simulink library "outp"  (R2021b)
(part 7 of 11)

      link override Signal_Limit/_minval: Value=KOUTP_LimpHomeActTmp_flg_minval
      link override Signal_Override/_ovrdflg: Value=KOUTP_LimpHomeActTmp_flg_ovrdflg
      link override Signal_Override/_ovrdval: Value=KOUTP_LimpHomeActTmp_flg_ovrdval
  VDDM_Lv1ErrDTC_raw32_Inproc : FVT_lib/outp/OverrideAndLimit  SystemSampleTime=-1  VariantActivationTime=update diagram  Latency=0  AutoFrameSizeCalculation=off
      link override Signal_Limit/_maxval: Value=KOUTP_Lv1ErrDTC_raw32_maxval
      link override Signal_Limit/_minval: Value=KOUTP_Lv1ErrDTC_raw32_minval
      link override Signal_Override/_ovrdflg: Value=KOUTP_Lv1ErrDTC_raw32_ovrdflg
      link override Signal_Override/_ovrdval: Value=KOUTP_Lv1ErrDTC_raw32_ovrdval
  VDDM_Lv2ErrDTC_raw32_Inproc : FVT_lib/outp/OverrideAndLimit  SystemSampleTime=-1  VariantActivationTime=update diagram  Latency=0  AutoFrameSizeCalculation=off
      link override Signal_Limit/_maxval: Value=KOUTP_Lv2ErrDTC_raw32_maxval
      link override Signal_Limit/_minval: Value=KOUTP_Lv2ErrDTC_raw32_minval
      link override Signal_Override/_ovrdflg: Value=KOUTP_Lv2ErrDTC_raw32_ovrdflg
      link override Signal_Override/_ovrdval: Value=KOUTP_Lv2ErrDTC_raw32_ovrdval
  VDDM_Lv3ErrDTC_raw32_Inproc : FVT_lib/outp/OverrideAndLimit  SystemSampleTime=-1  VariantActivationTime=update diagram  Latency=0  AutoFrameSizeCalculation=off
      link override Signal_Limit/_maxval: Value=KOUTP_Lv3ErrDTC_raw32_maxval
      link override Signal_Limit/_minval: Value=KOUTP_Lv3ErrDTC_raw32_minval
      link override Signal_Override/_ovrdflg: Value=KOUTP_Lv3ErrDTC_raw32_ovrdflg
      link override Signal_Override/_ovrdval: Value=KOUTP_Lv3ErrDTC_raw32_ovrdval
  VDDM_Lv4ErrDTC_raw32_Inproc : FVT_lib/outp/OverrideAndLimit  SystemSampleTime=-1  VariantActivationTime=update diagram  Latency=0  AutoFrameSizeCalculation=off
      link override Signal_Limit/_maxval: Value=KOUTP_Lv4ErrDTC_raw32_maxval
      link override Signal_Limit/_minval: Value=KOUTP_Lv4ErrDTC_raw32_minval
      link override Signal_Override/_ovrdflg: Value=KOUTP_Lv4ErrDTC_raw32_ovrdflg
      link override Signal_Override/_ovrdval: Value=KOUTP_Lv4ErrDTC_raw32_ovrdval
  VDDM_MCU4PreDTC_raw32_Inproc : FVT_lib/outp/OverrideAndLimit  SystemSampleTime=-1  VariantActivationTime=update diagram  Latency=0  AutoFrameSizeCalculation=off
      link override Signal_Limit/_maxval: Value=KOUTP_MCU4PreDTC_raw32_maxval
      link override Signal_Limit/_minval: Value=KOUTP_MCU4PreDTC_raw32_minval
      link override Signal_Override/_ovrdflg: Value=KOUTP_MCU4PreDTC_raw32_ovrdflg
      link override Signal_Override/_ovrdval: Value=KOUTP_MCU4PreDTC_raw32_ovrdval
  VDDM_MCUActDTC_raw32_Inproc : FVT_lib/outp/OverrideAndLimit  SystemSampleTime=-1  VariantActivationTime=update diagram  Latency=0  AutoFrameSizeCalculation=off
      link override Signal_Limit/_maxval: Value=KOUTP_MCUActDTC_raw32_maxval
      link override Signal_Limit/_minval: Value=KOUTP_MCUActDTC_raw32_minval
      link override Signal_Override/_ovrdflg: Value=KOUTP_MCUActDTC_raw32_ovrdflg
      link override Signal_Override/_ovrdval: Value=KOUTP_MCUActDTC_raw32_ovrdval
  VDDM_MCUActDisFail_flg_Inproc : FVT_lib/outp/OverrideAndLimit  SystemSampleTime=-1  VariantActivationTime=update diagram  Latency=0  AutoFrameSizeCalculation=off
      link override Signal_Limit/_maxval: Value=KOUTP_MCUActDisFail_flg_maxval
      link override Signal_Limit/_minval: Value=KOUTP_MCUActDisFail_flg_minval
      link override Signal_Override/_ovrdflg: Value=KOUTP_MCUActDisFail_flg_ovrdflg
      link override Signal_Override/_ovrdval: Value=KOUTP_MCUActDisFail_flg_ovrdval
  VDDM_MCUDisDTC_raw32_Inproc : FVT_lib/outp/OverrideAndLimit  SystemSampleTime=-1  VariantActivationTime=update diagram  Latency=0  AutoFrameSizeCalculation=off
      link override Signal_Limit/_maxval: Value=KOUTP_MCUDisDTC_raw32_maxval
      link override Signal_Limit/_minval: Value=KOUTP_MCUDisDTC_raw32_minval
      link override Signal_Override/_ovrdflg: Value=KOUTP_MCUDisDTC_raw32_ovrdflg
      link override Signal_Override/_ovrdval: Value=KOUTP_MCUDisDTC_raw32_ovrdval
  VDDM_MCUF1CSErrDTC_raw32_Inproc : FVT_lib/outp/OverrideAndLimit  SystemSampleTime=-1  VariantActivationTime=update diagram  Latency=0  AutoFrameSizeCalculation=off
      link override Signal_Limit/_maxval: Value=KOUTP_MCUF1CSErrDTC_raw32_maxval
      link override Signal_Limit/_minval: Value=KOUTP_MCUF1CSErrDTC_raw32_minval
      link override Signal_Override/_ovrdflg: Value=KOUTP_MCUF1CSErrDTC_raw32_ovrdflg
      link override Signal_Override/_ovrdval: Value=KOUTP_MCUF1CSErrDTC_raw32_ovrdval
  VDDM_MCUF1NoComDTC_raw32_Inproc : FVT_lib/outp/OverrideAndLimit  SystemSampleTime=-1  VariantActivationTime=update diagram  Latency=0  AutoFrameSizeCalculation=off
      link override Signal_Limit/_maxval: Value=KOUTP_MCUF1NoComDTC_raw32_maxval
      link override Signal_Limit/_minval: Value=KOUTP_MCUF1NoComDTC_raw32_minval
      link override Signal_Override/_ovrdflg: Value=KOUTP_MCUF1NoComDTC_raw32_ovrdflg
      link override Signal_Override/_ovrdval: Value=KOUTP_MCUF1NoComDTC_raw32_ovrdval
  VDDM_MCUF1RCErrDTC_raw32_Inproc : FVT_lib/outp/OverrideAndLimit  SystemSampleTime=-1  VariantActivationTime=update diagram  Latency=0  AutoFrameSizeCalculation=off
      link override Signal_Limit/_maxval: Value=KOUTP_MCUF1RCErrDTC_raw32_maxval
      link override Signal_Limit/_minval: Value=KOUTP_MCUF1RCErrDTC_raw32_minval
      link override Signal_Override/_ovrdflg: Value=KOUTP_MCUF1RCErrDTC_raw32_ovrdflg
      link override Signal_Override/_ovrdval: Value=KOUTP_MCUF1RCErrDTC_raw32_ovrdval
  VDDM_MCUR1CSErrDTC_raw32_Inproc : FVT_lib/outp/OverrideAndLimit  SystemSampleTime=-1  VariantActivationTime=update diagram  Latency=0  AutoFrameSizeCalculation=off
      link override Signal_Limit/_maxval: Value=KOUTP_MCUR1CSErrDTC_raw32_maxval
      link override Signal_Limit/_minval: Value=KOUTP_MCUR1CSErrDTC_raw32_minval
      link override Signal_Override/_ovrdflg: Value=KOUTP_MCUR1CSErrDTC_raw32_ovrdflg
      link override Signal_Override/_ovrdval: Value=KOUTP_MCUR1CSErrDTC_raw32_ovrdval
  VDDM_MCUR1NoComDTC_raw32_Inproc : FVT_lib/outp/OverrideAndLimit  SystemSampleTime=-1  VariantActivationTime=update diagram  Latency=0  AutoFrameSizeCalculation=off
      link override Signal_Limit/_maxval: Value=KOUTP_MCUR1NoComDTC_raw32_maxval
      link override Signal_Limit/_minval: Value=KOUTP_MCUR1NoComDTC_raw32_minval
      link override Signal_Override/_ovrdflg: Value=KOUTP_MCUR1NoComDTC_raw32_ovrdflg
      link override Signal_Override/_ovrdval: Value=KOUTP_MCUR1NoComDTC_raw32_ovrdval
  VDDM_MCUR1RCErrDTC_raw32_Inproc : FVT_lib/outp/OverrideAndLimit  SystemSampleTime=-1  VariantActivationTime=update diagram  Latency=0  AutoFrameSizeCalculation=off
      link override Signal_Limit/_maxval: Value=KOUTP_MCUR1RCErrDTC_raw32_maxval
      link override Signal_Limit/_minval: Value=KOUTP_MCUR1RCErrDTC_raw32_minval
      link override Signal_Override/_ovrdflg: Value=KOUTP_MCUR1RCErrDTC_raw32_ovrdflg
      link override Signal_Override/_ovrdval: Value=KOUTP_MCUR1RCErrDTC_raw32_ovrdval
  VDDM_MSAMalfuncDetDTC_raw32_Inproc : FVT_lib/outp/OverrideAndLimit  SystemSampleTime=-1  VariantActivationTime=update diagram  Latency=0  AutoFrameSizeCalculation=off
      link override Signal_Limit/_maxval: Value=KOUTP_MSAMalfuncDetDTC_raw32_maxval
      link override Signal_Limit/_minval: Value=KOUTP_MSAMalfuncDetDTC_raw32_minval
      link override Signal_Override/_ovrdflg: Value=KOUTP_MSAMalfuncDetDTC_raw32_ovrdflg
      link override Signal_Override/_ovrdval: Value=KOUTP_MSAMalfuncDetDTC_raw32_ovrdval
  VDDM_MidLvSaChkDTC_raw32_Inproc : FVT_lib/outp/OverrideAndLimit  SystemSampleTime=-1  VariantActivationTime=update diagram  Latency=0  AutoFrameSizeCalculation=off
      link override Signal_Limit/_maxval: Value=KOUTP_MidLvSaChkDTC_raw32_maxval
      link override Signal_Limit/_minval: Value=KOUTP_MidLvSaChkDTC_raw32_minval
      link override Signal_Override/_ovrdflg: Value=KOUTP_MidLvSaChkDTC_raw32_ovrdflg
      link override Signal_Override/_ovrdval: Value=KOUTP_MidLvSaChkDTC_raw32_ovrdval
  VDDM_OBC4PreDTC_raw32_Inproc : FVT_lib/outp/OverrideAndLimit  SystemSampleTime=-1  VariantActivationTime=update diagram  Latency=0  AutoFrameSizeCalculation=off
      link override Signal_Limit/_maxval: Value=KOUTP_OBC4PreDTC_raw32_maxval
      link override Signal_Limit/_minval: Value=KOUTP_OBC4PreDTC_raw32_minval
      link override Signal_Override/_ovrdflg: Value=KOUTP_OBC4PreDTC_raw32_ovrdflg
      link override Signal_Override/_ovrdval: Value=KOUTP_OBC4PreDTC_raw32_ovrdval
  VDDM_ONtoRdyDTC_raw32_Inproc : FVT_lib/outp/OverrideAndLimit  SystemSampleTime=-1  VariantActivationTime=update diagram  Latency=0  AutoFrameSizeCalculation=off
      link override Signal_Limit/_maxval: Value=KOUTP_ONtoRdyDTC_raw32_maxval
      link override Signal_Limit/_minval: Value=KOUTP_ONtoRdyDTC_raw32_minval
      link override Signal_Override/_ovrdflg: Value=KOUTP_ONtoRdyDTC_raw32_ovrdflg
      link override Signal_Override/_ovrdval: Value=KOUTP_ONtoRdyDTC_raw32_ovrdval
  VDDM_RCLUSSDTC_raw32_Inproc : FVT_lib/outp/OverrideAndLimit  SystemSampleTime=-1  VariantActivationTime=update diagram  Latency=0  AutoFrameSizeCalculation=off
      link override Signal_Limit/_maxval: Value=KOUTP_RCLUSSDTC_raw32_maxval
      link override Signal_Limit/_minval: Value=KOUTP_RCLUSSDTC_raw32_minval
      link override Signal_Override/_ovrdflg: Value=KOUTP_RCLUSSDTC_raw32_ovrdflg
      link override Signal_Override/_ovrdval: Value=KOUTP_RCLUSSDTC_raw32_ovrdval
  VDDM_RCRUSSDTC_raw32_Inproc : FVT_lib/outp/OverrideAndLimit  SystemSampleTime=-1  VariantActivationTime=update diagram  Latency=0  AutoFrameSizeCalculation=off
      link override Signal_Limit/_maxval: Value=KOUTP_RCRUSSDTC_raw32_maxval
      link override Signal_Limit/_minval: Value=KOUTP_RCRUSSDTC_raw32_minval
      link override Signal_Override/_ovrdflg: Value=KOUTP_RCRUSSDTC_raw32_ovrdflg
      link override Signal_Override/_ovrdval: Value=KOUTP_RCRUSSDTC_raw32_ovrdval
  VDDM_RFBatwarnDTC_raw32_Inproc : FVT_lib/outp/OverrideAndLimit  SystemSampleTime=-1  VariantActivationTime=update diagram  Latency=0  AutoFrameSizeCalculation=off
      link override Signal_Limit/_maxval: Value=KOUTP_RFBatwarnDTC_raw32_maxval
      link override Signal_Limit/_minval: Value=KOUTP_RFBatwarnDTC_raw32_minval
      link override Signal_Override/_ovrdflg: Value=KOUTP_RFBatwarnDTC_raw32_ovrdflg
      link override Signal_Override/_ovrdval: Value=KOUTP_RFBatwarnDTC_raw32_ovrdval
  VDDM_RFPressIndiDTC_raw32_Inproc : FVT_lib/outp/OverrideAndLimit  SystemSampleTime=-1  VariantActivationTime=update diagram  Latency=0  AutoFrameSizeCalculation=off
      link override Signal_Limit/_maxval: Value=KOUTP_RFPressIndiDTC_raw32_maxval
      link override Signal_Limit/_minval: Value=KOUTP_RFPressIndiDTC_raw32_minval
      link override Signal_Override/_ovrdflg: Value=KOUTP_RFPressIndiDTC_raw32_ovrdflg
      link override Signal_Override/_ovrdval: Value=KOUTP_RFPressIndiDTC_raw32_ovrdval
  VDDM_RFSensorFailDTC_raw32_Inproc : FVT_lib/outp/OverrideAndLimit  SystemSampleTime=-1  VariantActivationTime=update diagram  Latency=0  AutoFrameSizeCalculation=off
      link override Signal_Limit/_maxval: Value=KOUTP_RFSensorFailDTC_raw32_maxval
      link override Signal_Limit/_minval: Value=KOUTP_RFSensorFailDTC_raw32_minval
      link override Signal_Override/_ovrdflg: Value=KOUTP_RFSensorFailDTC_raw32_ovrdflg
      link override Signal_Override/_ovrdval: Value=KOUTP_RFSensorFailDTC_raw32_ovrdval
  VDDM_RFWheelTmpHighDTC_raw32_Inproc : FVT_lib/outp/OverrideAndLimit  SystemSampleTime=-1  VariantActivationTime=update diagram  Latency=0  AutoFrameSizeCalculation=off
      link override Signal_Limit/_maxval: Value=KOUTP_RFWheelTmpHighDTC_raw32_maxval
      link override Signal_Limit/_minval: Value=KOUTP_RFWheelTmpHighDTC_raw32_minval
      link override Signal_Override/_ovrdflg: Value=KOUTP_RFWheelTmpHighDTC_raw32_ovrdflg
      link override Signal_Override/_ovrdval: Value=KOUTP_RFWheelTmpHighDTC_raw32_ovrdval
  VDDM_RLDoorSWDTC_raw32_Inproc : FVT_lib/outp/OverrideAndLimit  SystemSampleTime=-1  VariantActivationTime=update diagram  Latency=0  AutoFrameSizeCalculation=off
      link override Signal_Limit/_maxval: Value=KOUTP_RLDoorSWDTC_raw32_maxval
      link override Signal_Limit/_minval: Value=KOUTP_RLDoorSWDTC_raw32_minval
      link override Signal_Override/_ovrdflg: Value=KOUTP_RLDoorSWDTC_raw32_ovrdflg
      link override Signal_Override/_ovrdval: Value=KOUTP_RLDoorSWDTC_raw32_ovrdval
  VDDM_RLLUSSDTC_raw32_Inproc : FVT_lib/outp/OverrideAndLimit  SystemSampleTime=-1  VariantActivationTime=update diagram  Latency=0  AutoFrameSizeCalculation=off
      link override Signal_Limit/_maxval: Value=KOUTP_RLLUSSDTC_raw32_maxval
      link override Signal_Limit/_minval: Value=KOUTP_RLLUSSDTC_raw32_minval
      link override Signal_Override/_ovrdflg: Value=KOUTP_RLLUSSDTC_raw32_ovrdflg
      link override Signal_Override/_ovrdval: Value=KOUTP_RLLUSSDTC_raw32_ovrdval
  VDDM_RLRUSSDTC_raw32_Inproc : FVT_lib/outp/OverrideAndLimit  SystemSampleTime=-1  VariantActivationTime=update diagram  Latency=0  AutoFrameSizeCalculation=off
      link override Signal_Limit/_maxval: Value=KOUTP_RLRUSSDTC_raw32_maxval
      link override Signal_Limit/_minval: Value=KOUTP_RLRUSSDTC_raw32_minval
      link override Signal_Override/_ovrdflg: Value=KOUTP_RLRUSSDTC_raw32_ovrdflg
      link override Signal_Override/_ovrdval: Value=KOUTP_RLRUSSDTC_raw32_ovrdval
  VDDM_RMLUSSDTC_raw32_Inproc : FVT_lib/outp/OverrideAndLimit  SystemSampleTime=-1  VariantActivationTime=update diagram  Latency=0  AutoFrameSizeCalculation=off
      link override Signal_Limit/_maxval: Value=KOUTP_RMLUSSDTC_raw32_maxval
      link override Signal_Limit/_minval: Value=KOUTP_RMLUSSDTC_raw32_minval
      link override Signal_Override/_ovrdflg: Value=KOUTP_RMLUSSDTC_raw32_ovrdflg
      link override Signal_Override/_ovrdval: Value=KOUTP_RMLUSSDTC_raw32_ovrdval
  VDDM_RMRUSSDTC_raw32_Inproc : FVT_lib/outp/OverrideAndLimit  SystemSampleTime=-1  VariantActivationTime=update diagram  Latency=0  AutoFrameSizeCalculation=off
      link override Signal_Limit/_maxval: Value=KOUTP_RMRUSSDTC_raw32_maxval
      link override Signal_Limit/_minval: Value=KOUTP_RMRUSSDTC_raw32_minval
      link override Signal_Override/_ovrdflg: Value=KOUTP_RMRUSSDTC_raw32_ovrdflg
      link override Signal_Override/_ovrdval: Value=KOUTP_RMRUSSDTC_raw32_ovrdval
  VDDM_RRBatwarnDTC_raw32_Inproc : FVT_lib/outp/OverrideAndLimit  SystemSampleTime=-1  VariantActivationTime=update diagram  Latency=0  AutoFrameSizeCalculation=off
      link override Signal_Limit/_maxval: Value=KOUTP_RRBatwarnDTC_raw32_maxval
      link override Signal_Limit/_minval: Value=KOUTP_RRBatwarnDTC_raw32_minval
      link override Signal_Override/_ovrdflg: Value=KOUTP_RRBatwarnDTC_raw32_ovrdflg
      link override Signal_Override/_ovrdval: Value=KOUTP_RRBatwarnDTC_raw32_ovrdval
  VDDM_RRDoorSWDTC_raw32_Inproc : FVT_lib/outp/OverrideAndLimit  SystemSampleTime=-1  VariantActivationTime=update diagram  Latency=0  AutoFrameSizeCalculation=off
      link override Signal_Limit/_maxval: Value=KOUTP_RRDoorSWDTC_raw32_maxval
      link override Signal_Limit/_minval: Value=KOUTP_RRDoorSWDTC_raw32_minval
      link override Signal_Override/_ovrdflg: Value=KOUTP_RRDoorSWDTC_raw32_ovrdflg
      link override Signal_Override/_ovrdval: Value=KOUTP_RRDoorSWDTC_raw32_ovrdval
  VDDM_RRPressIndiDTC_raw32_Inproc : FVT_lib/outp/OverrideAndLimit  SystemSampleTime=-1  VariantActivationTime=update diagram  Latency=0  AutoFrameSizeCalculation=off
      link override Signal_Limit/_maxval: Value=KOUTP_RRPressIndiDTC_raw32_maxval
      link override Signal_Limit/_minval: Value=KOUTP_RRPressIndiDTC_raw32_minval
      link override Signal_Override/_ovrdflg: Value=KOUTP_RRPressIndiDTC_raw32_ovrdflg
      link override Signal_Override/_ovrdval: Value=KOUTP_RRPressIndiDTC_raw32_ovrdval
  VDDM_RRSensorFailDTC_raw32_Inproc : FVT_lib/outp/OverrideAndLimit  SystemSampleTime=-1  VariantActivationTime=update diagram  Latency=0  AutoFrameSizeCalculation=off
      link override Signal_Limit/_maxval: Value=KOUTP_RRSensorFailDTC_raw32_maxval
      link override Signal_Limit/_minval: Value=KOUTP_RRSensorFailDTC_raw32_minval
      link override Signal_Override/_ovrdflg: Value=KOUTP_RRSensorFailDTC_raw32_ovrdflg
      link override Signal_Override/_ovrdval: Value=KOUTP_RRSensorFailDTC_raw32_ovrdval
  VDDM_RRWheelTmpHighDTC_raw32_Inproc : FVT_lib/outp/OverrideAndLimit  SystemSampleTime=-1  VariantActivationTime=update diagram  Latency=0  AutoFrameSizeCalculation=off
      link override Signal_Limit/_maxval: Value=KOUTP_RRWheelTmpHighDTC_raw32_maxval
      link override Signal_Limit/_minval: Value=KOUTP_RRWheelTmpHighDTC_raw32_minval
      link override Signal_Override/_ovrdflg: Value=KOUTP_RRWheelTmpHighDTC_raw32_ovrdflg
      link override Signal_Override/_ovrdval: Value=KOUTP_RRWheelTmpHighDTC_raw32_ovrdval
  VDDM_RrMCUSigErrDetDTC_raw32_Inproc : FVT_lib/outp/OverrideAndLimit  SystemSampleTime=-1  VariantActivationTime=update diagram  Latency=0  AutoFrameSizeCalculation=off
      link override Signal_Limit/_maxval: Value=KOUTP_RrMCUSigErrDetDTC_raw32_maxval
      link override Signal_Limit/_minval: Value=KOUTP_RrMCUSigErrDetDTC_raw32_minval
      link override Signal_Override/_ovrdflg: Value=KOUTP_RrMCUSigErrDetDTC_raw32_ovrdflg
      link override Signal_Override/_ovrdval: Value=KOUTP_RrMCUSigErrDetDTC_raw32_ovrdval
  VDDM_RrMCUTqErrDTC_raw32_Inproc : FVT_lib/outp/OverrideAndLimit  SystemSampleTime=-1  VariantActivationTime=update diagram  Latency=0  AutoFrameSizeCalculation=off
      link override Signal_Limit/_maxval: Value=KOUTP_RrMCUTqErrDTC_raw32_maxval
      link override Signal_Limit/_minval: Value=KOUTP_RrMCUTqErrDTC_raw32_minval
      link override Signal_Override/_ovrdflg: Value=KOUTP_RrMCUTqErrDTC_raw32_ovrdflg
      link override Signal_Override/_ovrdval: Value=KOUTP_RrMCUTqErrDTC_raw32_ovrdval
  VDDM_Shifter1CSErrDTC_raw32_Inproc : FVT_lib/outp/OverrideAndLimit  SystemSampleTime=-1  VariantActivationTime=update diagram  Latency=0  AutoFrameSizeCalculation=off
      link override Signal_Limit/_maxval: Value=KOUTP_Shifter1CSErrDTC_raw32_maxval
      link override Signal_Limit/_minval: Value=KOUTP_Shifter1CSErrDTC_raw32_minval
      link override Signal_Override/_ovrdflg: Value=KOUTP_Shifter1CSErrDTC_raw32_ovrdflg
      link override Signal_Override/_ovrdval: Value=KOUTP_Shifter1CSErrDTC_raw32_ovrdval
  VDDM_Shifter1NoComDTC_raw32_Inproc : FVT_lib/outp/OverrideAndLimit  SystemSampleTime=-1  VariantActivationTime=update diagram  Latency=0  AutoFrameSizeCalculation=off
      link override Signal_Limit/_maxval: Value=KOUTP_Shifter1NoComDTC_raw32_maxval
      link override Signal_Limit/_minval: Value=KOUTP_Shifter1NoComDTC_raw32_minval
      link override Signal_Override/_ovrdflg: Value=KOUTP_Shifter1NoComDTC_raw32_ovrdflg
      link override Signal_Override/_ovrdval: Value=KOUTP_Shifter1NoComDTC_raw32_ovrdval
  VDDM_Shifter1RCErrDTC_raw32_Inproc : FVT_lib/outp/OverrideAndLimit  SystemSampleTime=-1  VariantActivationTime=update diagram  Latency=0  AutoFrameSizeCalculation=off
      link override Signal_Limit/_maxval: Value=KOUTP_Shifter1RCErrDTC_raw32_maxval
      link override Signal_Limit/_minval: Value=KOUTP_Shifter1RCErrDTC_raw32_minval
      link override Signal_Override/_ovrdflg: Value=KOUTP_Shifter1RCErrDTC_raw32_ovrdflg
      link override Signal_Override/_ovrdval: Value=KOUTP_Shifter1RCErrDTC_raw32_ovrdval
  VDDM_SysAllowReadySta_flg_Inproc : FVT_lib/outp/OverrideAndLimit  SystemSampleTime=-1  VariantActivationTime=update diagram  Latency=0  AutoFrameSizeCalculation=off
      link override Signal_Limit/_maxval: Value=KOUTP_SysAllowReadySta_flg_maxval
      link override Signal_Limit/_minval: Value=KOUTP_SysAllowReadySta_flg_minval
      link override Signal_Override/_ovrdflg: Value=KOUTP_SysAllowReadySta_flg_ovrdflg
      link override Signal_Override/_ovrdval: Value=KOUTP_SysAllowReadySta_flg_ovrdval
  VDDM_TailgaSWDTC_raw32_Inproc : FVT_lib/outp/OverrideAndLimit  SystemSampleTime=-1  VariantActivationTime=update diagram  Latency=0  AutoFrameSizeCalculation=off
      link override Signal_Limit/_maxval: Value=KOUTP_TailgaSWDTC_raw32_maxval
      link override Signal_Limit/_minval: Value=KOUTP_TailgaSWDTC_raw32_minval
      link override Signal_Override/_ovrdflg: Value=KOUTP_TailgaSWDTC_raw32_ovrdflg
      link override Signal_Override/_ovrdval: Value=KOUTP_TailgaSWDTC_raw32_ovrdval
  VDDM_VCUBrkSWSta_enum_Inproc : FVT_lib/outp/OverrideAndLimit  SystemSampleTime=-1  VariantActivationTime=update diagram  Latency=0  AutoFrameSizeCalculation=off
      link override Signal_Limit/_maxval: Value=KOUTP_VCUBrkSWSta_enum_maxval
      link override Signal_Limit/_minval: Value=KOUTP_VCUBrkSWSta_enum_minval
      link override Signal_Override/_ovrdflg: Value=KOUTP_VCUBrkSWSta_enum_ovrdflg
      link override Signal_Override/_ovrdval: Value=KOUTP_VCUBrkSWSta_enum_ovrdval
  VDDM_VCUFLDoorSta_flg_Inproc : FVT_lib/outp/OverrideAndLimit  SystemSampleTime=-1  VariantActivationTime=update diagram  Latency=0  AutoFrameSizeCalculation=off
      link override Signal_Limit/_maxval: Value=KOUTP_VCUFLDoorSta_flg_maxval
      link override Signal_Limit/_minval: Value=KOUTP_VCUFLDoorSta_flg_minval
      link override Signal_Override/_ovrdflg: Value=KOUTP_VCUFLDoorSta_flg_ovrdflg
      link override Signal_Override/_ovrdval: Value=KOUTP_VCUFLDoorSta_flg_ovrdval
  VDDM_VCUFRDoorSta_flg_Inproc : FVT_lib/outp/OverrideAndLimit  SystemSampleTime=-1  VariantActivationTime=update diagram  Latency=0  AutoFrameSizeCalculation=off
      link override Signal_Limit/_maxval: Value=KOUTP_VCUFRDoorSta_flg_maxval
      link override Signal_Limit/_minval: Value=KOUTP_VCUFRDoorSta_flg_minval
      link override Signal_Override/_ovrdflg: Value=KOUTP_VCUFRDoorSta_flg_ovrdflg
      link override Signal_Override/_ovrdval: Value=KOUTP_VCUFRDoorSta_flg_ovrdval
  VDDM_VCUHoodSWSta_flg_Inproc : FVT_lib/outp/OverrideAndLimit  SystemSampleTime=-1  VariantActivationTime=update diagram  Latency=0  AutoFrameSizeCalculation=off
      link override Signal_Limit/_maxval: Value=KOUTP_VCUHoodSWSta_flg_maxval
      link override Signal_Limit/_minval: Value=KOUTP_VCUHoodSWSta_flg_minval
      link override Signal_Override/_ovrdflg: Value=KOUTP_VCUHoodSWSta_flg_ovrdflg
      link override Signal_Override/_ovrdval: Value=KOUTP_VCUHoodSWSta_flg_ovrdval
  VDDM_VCURAPSErrLv2_flg_Inproc : FVT_lib/outp/OverrideAndLimit  SystemSampleTime=-1  VariantActivationTime=update diagram  Latency=0  AutoFrameSizeCalculation=off
      link override Signal_Limit/_maxval: Value=KOUTP_VCURAPSErrLv2_flg_maxval
      link override Signal_Limit/_minval: Value=KOUTP_VCURAPSErrLv2_flg_minval
      link override Signal_Override/_ovrdflg: Value=KOUTP_VCURAPSErrLv2_flg_ovrdflg
      link override Signal_Override/_ovrdval: Value=KOUTP_VCURAPSErrLv2_flg_ovrdval
  VDDM_VCURAPSErrLv3_flg_Inproc : FVT_lib/outp/OverrideAndLimit  SystemSampleTime=-1  VariantActivationTime=update diagram  Latency=0  AutoFrameSizeCalculation=off
      link override Signal_Limit/_maxval: Value=KOUTP_VCURAPSErrLv3_flg_maxval
      link override Signal_Limit/_minval: Value=KOUTP_VCURAPSErrLv3_flg_minval
      link override Signal_Override/_ovrdflg: Value=KOUTP_VCURAPSErrLv3_flg_ovrdflg
      link override Signal_Override/_ovrdval: Value=KOUTP_VCURAPSErrLv3_flg_ovrdval
  VDDM_VCURLDoorSta_flg_Inproc : FVT_lib/outp/OverrideAndLimit  SystemSampleTime=-1  VariantActivationTime=update diagram  Latency=0  AutoFrameSizeCalculation=off
      link override Signal_Limit/_maxval: Value=KOUTP_VCURLDoorSta_flg_maxval
      link override Signal_Limit/_minval: Value=KOUTP_VCURLDoorSta_flg_minval
      link override Signal_Override/_ovrdflg: Value=KOUTP_VCURLDoorSta_flg_ovrdflg
      link override Signal_Override/_ovrdval: Value=KOUTP_VCURLDoorSta_flg_ovrdval
  VDDM_VCURRDoorSta_flg_Inproc : FVT_lib/outp/OverrideAndLimit  SystemSampleTime=-1  VariantActivationTime=update diagram  Latency=0  AutoFrameSizeCalculation=off
      link override Signal_Limit/_maxval: Value=KOUTP_VCURRDoorSta_flg_maxval
      link override Signal_Limit/_minval: Value=KOUTP_VCURRDoorSta_flg_minval
      link override Signal_Override/_ovrdflg: Value=KOUTP_VCURRDoorSta_flg_ovrdflg
      link override Signal_Override/_ovrdval: Value=KOUTP_VCURRDoorSta_flg_ovrdval
  VDDM_VCUTailgateSWSta_flg_Inproc : FVT_lib/outp/OverrideAndLimit  SystemSampleTime=-1  VariantActivationTime=update diagram  Latency=0  AutoFrameSizeCalculation=off
      link override Signal_Limit/_maxval: Value=KOUTP_VCUTailgateSWSta_flg_maxval
      link override Signal_Limit/_minval: Value=KOUTP_VCUTailgateSWSta_flg_minval
      link override Signal_Override/_ovrdflg: Value=KOUTP_VCUTailgateSWSta_flg_ovrdflg
      link override Signal_Override/_ovrdval: Value=KOUTP_VCUTailgateSWSta_flg_ovrdval
  VDDM_VehMalfunLevel_enum_Inproc : FVT_lib/outp/OverrideAndLimit  SystemSampleTime=-1  VariantActivationTime=update diagram  Latency=0  AutoFrameSizeCalculation=off
      link override Signal_Limit/_maxval: Value=KOUTP_VehMalfunLevel_enum_maxval
      link override Signal_Limit/_minval: Value=KOUTP_VehMalfunLevel_enum_minval
      link override Signal_Override/_ovrdflg: Value=KOUTP_VehMalfunLevel_enum_ovrdflg
      link override Signal_Override/_ovrdval: Value=KOUTP_VehMalfunLevel_enum_ovrdval
  VDDM_ZoneSCPNoComDTC_raw32_Inproc : FVT_lib/outp/OverrideAndLimit  SystemSampleTime=-1  VariantActivationTime=update diagram  Latency=0  AutoFrameSizeCalculation=off
      link override Signal_Limit/_maxval: Value=KOUTP_ZoneSCPNoComDTC_raw32_maxval
      link override Signal_Limit/_minval: Value=KOUTP_ZoneSCPNoComDTC_raw32_minval
      link override Signal_Override/_ovrdflg: Value=KOUTP_ZoneSCPNoComDTC_raw32_ovrdflg
      link override Signal_Override/_ovrdval: Value=KOUTP_ZoneSCPNoComDTC_raw32_ovrdval
  VDHP_ActAPSPosn_pct_Inproc : FVT_lib/outp/OverrideAndLimit  SystemSampleTime=-1  VariantActivationTime=update diagram  Latency=0  AutoFrameSizeCalculation=off
      link override Signal_Limit/_maxval: Value=KOUTP_ActAPSPosn_pct_maxval
      link override Signal_Limit/_minval: Value=KOUTP_ActAPSPosn_pct_minval
      link override Signal_Override/_ovrdflg: Value=KOUTP_ActAPSPosn_pct_ovrdflg
      link override Signal_Override/_ovrdval: Value=KOUTP_ActAPSPosn_pct_ovrdval
  VDHP_EAPS1MIN_pct_Inproc : FVT_lib/outp/OverrideAndLimit  SystemSampleTime=-1  VariantActivationTime=update diagram  Latency=0  AutoFrameSizeCalculation=off
      link override Signal_Limit/_maxval: Value=KOUTP_EAPS1MIN_pct_maxval
      link override Signal_Limit/_minval: Value=KOUTP_EAPS1MIN_pct_minval
      link override Signal_Override/_ovrdflg: Value=KOUTP_EAPS1MIN_pct_ovrdflg
      link override Signal_Override/_ovrdval: Value=KOUTP_EAPS1MIN_pct_ovrdval
  VDHP_EAPS1NRM_pct_Inproc : FVT_lib/outp/OverrideAndLimit  SystemSampleTime=-1  VariantActivationTime=update diagram  Latency=0  AutoFrameSizeCalculation=off
      link override Signal_Limit/_maxval: Value=KOUTP_EAPS1NRM_pct_maxval
      link override Signal_Limit/_minval: Value=KOUTP_EAPS1NRM_pct_minval
      link override Signal_Override/_ovrdflg: Value=KOUTP_EAPS1NRM_pct_ovrdflg
      link override Signal_Override/_ovrdval: Value=KOUTP_EAPS1NRM_pct_ovrdval
  VDHP_EAPS2MIN_pct_Inproc : FVT_lib/outp/OverrideAndLimit  SystemSampleTime=-1  VariantActivationTime=update diagram  Latency=0  AutoFrameSizeCalculation=off
      link override Signal_Limit/_maxval: Value=KOUTP_EAPS2MIN_pct_maxval
      link override Signal_Limit/_minval: Value=KOUTP_EAPS2MIN_pct_minval
      link override Signal_Override/_ovrdflg: Value=KOUTP_EAPS2MIN_pct_ovrdflg
      link override Signal_Override/_ovrdval: Value=KOUTP_EAPS2MIN_pct_ovrdval
  VDHP_EAPS2NRM_pct_Inproc : FVT_lib/outp/OverrideAndLimit  SystemSampleTime=-1  VariantActivationTime=update diagram  Latency=0  AutoFrameSizeCalculation=off
      link override Signal_Limit/_maxval: Value=KOUTP_EAPS2NRM_pct_maxval
      link override Signal_Limit/_minval: Value=KOUTP_EAPS2NRM_pct_minval
      link override Signal_Override/_ovrdflg: Value=KOUTP_EAPS2NRM_pct_ovrdflg
      link override Signal_Override/_ovrdval: Value=KOUTP_EAPS2NRM_pct_ovrdval
  VDHP_ResetPedalZeroPosStart_flg_Inproc : FVT_lib/outp/OverrideAndLimit  SystemSampleTime=-1  VariantActivationTime=update diagram  Latency=0  AutoFrameSizeCalculation=off
      link override Signal_Limit/_maxval: Value=KOUTP_ResetPedalZeroPosStart_flg_maxval
      link override Signal_Limit/_minval: Value=KOUTP_ResetPedalZeroPosStart_flg_minval
      link override Signal_Override/_ovrdflg: Value=KOUTP_ResetPedalZeroPosStart_flg_ovrdflg
      link override Signal_Override/_ovrdval: Value=KOUTP_ResetPedalZeroPosStart_flg_ovrdval
  VDKC_DKCAuthSta_enum_Inproc : FVT_lib/outp/OverrideAndLimit  SystemSampleTime=-1  VariantActivationTime=update diagram  Latency=0  AutoFrameSizeCalculation=off
      link override Signal_Limit/_maxval: Value=KOUTP_DKCAuthSta_enum_maxval
      link override Signal_Limit/_minval: Value=KOUTP_DKCAuthSta_enum_minval
      link override Signal_Override/_ovrdflg: Value=KOUTP_DKCAuthSta_enum_ovrdflg
      link override Signal_Override/_ovrdval: Value=KOUTP_DKCAuthSta_enum_ovrdval
  VDKC_DKCTimeSN_cnt_Inproc : FVT_lib/outp/OverrideAndLimit  SystemSampleTime=-1  VariantActivationTime=update diagram  Latency=0  AutoFrameSizeCalculation=off
      link override Signal_Limit/_maxval: Value=KOUTP_DKCTimeSN_cnt_maxval
      link override Signal_Limit/_minval: Value=KOUTP_DKCTimeSN_cnt_minval
      link override Signal_Override/_ovrdflg: Value=KOUTP_DKCTimeSN_cnt_ovrdflg
      link override Signal_Override/_ovrdval: Value=KOUTP_DKCTimeSN_cnt_ovrdval
  VDKC_DKeyWelcomeSta_enum_Inproc : FVT_lib/outp/OverrideAndLimit  SystemSampleTime=-1  VariantActivationTime=update diagram  Latency=0  AutoFrameSizeCalculation=off
      link override Signal_Limit/_maxval: Value=KOUTP_DKeyWelcomeSta_enum_maxval
      link override Signal_Limit/_minval: Value=KOUTP_DKeyWelcomeSta_enum_minval
      link override Signal_Override/_ovrdflg: Value=KOUTP_DKeyWelcomeSta_enum_ovrdflg
      link override Signal_Override/_ovrdval: Value=KOUTP_DKeyWelcomeSta_enum_ovrdval
  VDKC_DkeyAreaRAPSSta_enum_Inproc : FVT_lib/outp/OverrideAndLimit  SystemSampleTime=-1  VariantActivationTime=update diagram  Latency=0  AutoFrameSizeCalculation=off
      link override Signal_Limit/_maxval: Value=KOUTP_DkeyAreaRAPSSta_enum_maxval
      link override Signal_Limit/_minval: Value=KOUTP_DkeyAreaRAPSSta_enum_minval
      link override Signal_Override/_ovrdflg: Value=KOUTP_DkeyAreaRAPSSta_enum_ovrdflg
      link override Signal_Override/_ovrdval: Value=KOUTP_DkeyAreaRAPSSta_enum_ovrdval
  VDKC_DkeyShowIVISta_enum_Inproc : FVT_lib/outp/OverrideAndLimit  SystemSampleTime=-1  VariantActivationTime=update diagram  Latency=0  AutoFrameSizeCalculation=off
      link override Signal_Limit/_maxval: Value=KOUTP_DkeyShowIVISta_enum_maxval
      link override Signal_Limit/_minval: Value=KOUTP_DkeyShowIVISta_enum_minval
      link override Signal_Override/_ovrdflg: Value=KOUTP_DkeyShowIVISta_enum_ovrdflg
      link override Signal_Override/_ovrdval: Value=KOUTP_DkeyShowIVISta_enum_ovrdval
  VDKC_FDCDKCAllowSleep_flg_Inproc : FVT_lib/outp/OverrideAndLimit  SystemSampleTime=-1  VariantActivationTime=update diagram  Latency=0  AutoFrameSizeCalculation=off
      link override Signal_Limit/_maxval: Value=KOUTP_FDCDKCAllowSleep_flg_maxval
      link override Signal_Limit/_minval: Value=KOUTP_FDCDKCAllowSleep_flg_minval
      link override Signal_Override/_ovrdflg: Value=KOUTP_FDCDKCAllowSleep_flg_ovrdflg
      link override Signal_Override/_ovrdval: Value=KOUTP_FDCDKCAllowSleep_flg_ovrdval
  VDKC_KeyAreaLockUnlock_enum_Inproc : FVT_lib/outp/OverrideAndLimit  SystemSampleTime=-1  VariantActivationTime=update diagram  Latency=0  AutoFrameSizeCalculation=off
      link override Signal_Limit/_maxval: Value=KOUTP_KeyAreaLockUnlock_enum_maxval
      link override Signal_Limit/_minval: Value=KOUTP_KeyAreaLockUnlock_enum_minval
      link override Signal_Override/_ovrdflg: Value=KOUTP_KeyAreaLockUnlock_enum_ovrdflg
      link override Signal_Override/_ovrdval: Value=KOUTP_KeyAreaLockUnlock_enum_ovrdval
  VDKC_KeyAreaPS_enum_Inproc : FVT_lib/outp/OverrideAndLimit  SystemSampleTime=-1  VariantActivationTime=update diagram  Latency=0  AutoFrameSizeCalculation=off
      link override Signal_Limit/_maxval: Value=KOUTP_KeyAreaPS_enum_maxval
      link override Signal_Limit/_minval: Value=KOUTP_KeyAreaPS_enum_minval
      link override Signal_Override/_ovrdflg: Value=KOUTP_KeyAreaPS_enum_ovrdflg
      link override Signal_Override/_ovrdval: Value=KOUTP_KeyAreaPS_enum_ovrdval
  VDKC_KeyAreaPTG_enum_Inproc : FVT_lib/outp/OverrideAndLimit  SystemSampleTime=-1  VariantActivationTime=update diagram  Latency=0  AutoFrameSizeCalculation=off
      link override Signal_Limit/_maxval: Value=KOUTP_KeyAreaPTG_enum_maxval
      link override Signal_Limit/_minval: Value=KOUTP_KeyAreaPTG_enum_minval
      link override Signal_Override/_ovrdflg: Value=KOUTP_KeyAreaPTG_enum_ovrdflg
      link override Signal_Override/_ovrdval: Value=KOUTP_KeyAreaPTG_enum_ovrdval
  VDKC_KeyAreaSPTGSta_enum_Inproc : FVT_lib/outp/OverrideAndLimit  SystemSampleTime=-1  VariantActivationTime=update diagram  Latency=0  AutoFrameSizeCalculation=off
      link override Signal_Limit/_maxval: Value=KOUTP_KeyAreaSPTGSta_enum_maxval
      link override Signal_Limit/_minval: Value=KOUTP_KeyAreaSPTGSta_enum_minval
      link override Signal_Override/_ovrdflg: Value=KOUTP_KeyAreaSPTGSta_enum_ovrdflg
      link override Signal_Override/_ovrdval: Value=KOUTP_KeyAreaSPTGSta_enum_ovrdval
  VDKC_KeyMissSta_flg_Inproc : FVT_lib/outp/OverrideAndLimit  SystemSampleTime=-1  VariantActivationTime=update diagram  Latency=0  AutoFrameSizeCalculation=off
      link override Signal_Limit/_maxval: Value=KOUTP_KeyMissSta_flg_maxval
      link override Signal_Limit/_minval: Value=KOUTP_KeyMissSta_flg_minval
      link override Signal_Override/_ovrdflg: Value=KOUTP_KeyMissSta_flg_ovrdflg
      link override Signal_Override/_ovrdval: Value=KOUTP_KeyMissSta_flg_ovrdval
  VDKC_KeyModeSta_enum_Inproc : FVT_lib/outp/OverrideAndLimit  SystemSampleTime=-1  VariantActivationTime=update diagram  Latency=0  AutoFrameSizeCalculation=off
      link override Signal_Limit/_maxval: Value=KOUTP_KeyModeSta_enum_maxval
      link override Signal_Limit/_minval: Value=KOUTP_KeyModeSta_enum_minval
      link override Signal_Override/_ovrdflg: Value=KOUTP_KeyModeSta_enum_ovrdflg
      link override Signal_Override/_ovrdval: Value=KOUTP_KeyModeSta_enum_ovrdval
  VDKC_KeyNumSta_enum_Inproc : FVT_lib/outp/OverrideAndLimit  SystemSampleTime=-1  VariantActivationTime=update diagram  Latency=0  AutoFrameSizeCalculation=off
      link override Signal_Limit/_maxval: Value=KOUTP_KeyNumSta_enum_maxval
      link override Signal_Limit/_minval: Value=KOUTP_KeyNumSta_enum_minval
      link override Signal_Override/_ovrdflg: Value=KOUTP_KeyNumSta_enum_ovrdflg
      link override Signal_Override/_ovrdval: Value=KOUTP_KeyNumSta_enum_ovrdval
  VDKC_KeyTypeSta_enum_Inproc : FVT_lib/outp/OverrideAndLimit  SystemSampleTime=-1  VariantActivationTime=update diagram  Latency=0  AutoFrameSizeCalculation=off
      link override Signal_Limit/_maxval: Value=KOUTP_KeyTypeSta_enum_maxval
      link override Signal_Limit/_minval: Value=KOUTP_KeyTypeSta_enum_minval
      link override Signal_Override/_ovrdflg: Value=KOUTP_KeyTypeSta_enum_ovrdflg
      link override Signal_Override/_ovrdval: Value=KOUTP_KeyTypeSta_enum_ovrdval
  VDKC_PCommandToBCM_enum_Inproc : FVT_lib/outp/OverrideAndLimit  SystemSampleTime=-1  VariantActivationTime=update diagram  Latency=0  AutoFrameSizeCalculation=off
      link override Signal_Limit/_maxval: Value=KOUTP_PCommandToBCM_enum_maxval
      link override Signal_Limit/_minval: Value=KOUTP_PCommandToBCM_enum_minval
      link override Signal_Override/_ovrdflg: Value=KOUTP_PCommandToBCM_enum_ovrdflg
      link override Signal_Override/_ovrdval: Value=KOUTP_PCommandToBCM_enum_ovrdval
  VDKC_ParkingModeCmd_enum_Inproc : FVT_lib/outp/OverrideAndLimit  SystemSampleTime=-1  VariantActivationTime=update diagram  Latency=0  AutoFrameSizeCalculation=off
      link override Signal_Limit/_maxval: Value=KOUTP_ParkingModeCmd_enum_maxval
      link override Signal_Limit/_minval: Value=KOUTP_ParkingModeCmd_enum_minval
      link override Signal_Override/_ovrdflg: Value=KOUTP_ParkingModeCmd_enum_ovrdflg
      link override Signal_Override/_ovrdval: Value=KOUTP_ParkingModeCmd_enum_ovrdval
  VDKC_TimeSNDKCFbk_cnt_Inproc : FVT_lib/outp/OverrideAndLimit  SystemSampleTime=-1  VariantActivationTime=update diagram  Latency=0  AutoFrameSizeCalculation=off
      link override Signal_Limit/_maxval: Value=KOUTP_TimeSNDKCFbk_cnt_maxval
      link override Signal_Limit/_minval: Value=KOUTP_TimeSNDKCFbk_cnt_minval
      link override Signal_Override/_ovrdflg: Value=KOUTP_TimeSNDKCFbk_cnt_ovrdflg
      link override Signal_Override/_ovrdval: Value=KOUTP_TimeSNDKCFbk_cnt_ovrdval
  VDKC_UIDLowPowerSta_enum_Inproc : FVT_lib/outp/OverrideAndLimit  SystemSampleTime=-1  VariantActivationTime=update diagram  Latency=0  AutoFrameSizeCalculation=off
      link override Signal_Limit/_maxval: Value=KOUTP_UIDLowPowerSta_enum_maxval
      link override Signal_Limit/_minval: Value=KOUTP_UIDLowPowerSta_enum_minval
      link override Signal_Override/_ovrdflg: Value=KOUTP_UIDLowPowerSta_enum_ovrdflg
      link override Signal_Override/_ovrdval: Value=KOUTP_UIDLowPowerSta_enum_ovrdval
  VDSC_DISCButtSta_flg_Inproc : FVT_lib/outp/OverrideAndLimit  SystemSampleTime=-1  VariantActivationTime=update diagram  Latency=0  AutoFrameSizeCalculation=off
      link override Signal_Limit/_maxval: Value=KOUTP_DISCButtSta_flg_maxval
      link override Signal_Limit/_minval: Value=KOUTP_DISCButtSta_flg_minval
      link override Signal_Override/_ovrdflg: Value=KOUTP_DISCButtSta_flg_ovrdflg
      link override Signal_Override/_ovrdval: Value=KOUTP_DISCButtSta_flg_ovrdval
  VDSC_DISCSta_enum_Inproc : FVT_lib/outp/OverrideAndLimit  SystemSampleTime=-1  VariantActivationTime=update diagram  Latency=0  AutoFrameSizeCalculation=off
      link override Signal_Limit/_maxval: Value=KOUTP_DISCSta_enum_maxval
      link override Signal_Limit/_minval: Value=KOUTP_DISCSta_enum_minval
      link override Signal_Override/_ovrdflg: Value=KOUTP_DISCSta_enum_ovrdflg
      link override Signal_Override/_ovrdval: Value=KOUTP_DISCSta_enum_ovrdval
  VDSC_DISCTargetSpd_kph_Inproc : FVT_lib/outp/OverrideAndLimit  SystemSampleTime=-1  VariantActivationTime=update diagram  Latency=0  AutoFrameSizeCalculation=off
      link override Signal_Limit/_maxval: Value=KOUTP_DISCTargetSpd_kph_maxval
      link override Signal_Limit/_minval: Value=KOUTP_DISCTargetSpd_kph_minval
      link override Signal_Override/_ovrdflg: Value=KOUTP_DISCTargetSpd_kph_ovrdflg
      link override Signal_Override/_ovrdval: Value=KOUTP_DISCTargetSpd_kph_ovrdval
  VDSC_DISCTurn_flg_Inproc : FVT_lib/outp/OverrideAndLimit  SystemSampleTime=-1  VariantActivationTime=update diagram  Latency=0  AutoFrameSizeCalculation=off
      link override Signal_Limit/_maxval: Value=KOUTP_DISCTurn_flg_maxval
      link override Signal_Limit/_minval: Value=KOUTP_DISCTurn_flg_minval
      link override Signal_Override/_ovrdflg: Value=KOUTP_DISCTurn_flg_ovrdflg
      link override Signal_Override/_ovrdval: Value=KOUTP_DISCTurn_flg_ovrdval
  VNMM_ActiveWU_flg_Inproc : FVT_lib/outp/OverrideAndLimit  SystemSampleTime=-1  VariantActivationTime=update diagram  Latency=0  AutoFrameSizeCalculation=off
      link override Signal_Limit/_maxval: Value=KOUTP_ActiveWU_flg_maxval
      link override Signal_Limit/_minval: Value=KOUTP_ActiveWU_flg_minval
      link override Signal_Override/_ovrdflg: Value=KOUTP_ActiveWU_flg_ovrdflg
      link override Signal_Override/_ovrdval: Value=KOUTP_ActiveWU_flg_ovrdval
  VNMM_AllCANTxReq_flg_Inproc : FVT_lib/outp/OverrideAndLimit  SystemSampleTime=-1  VariantActivationTime=update diagram  Latency=0  AutoFrameSizeCalculation=off
      link override Signal_Limit/_maxval: Value=KOUTP_AllCANTxReq_flg_maxval
      link override Signal_Limit/_minval: Value=KOUTP_AllCANTxReq_flg_minval
      link override Signal_Override/_ovrdflg: Value=KOUTP_AllCANTxReq_flg_ovrdflg
      link override Signal_Override/_ovrdval: Value=KOUTP_AllCANTxReq_flg_ovrdval
  VNMM_Awake_enum_Inproc : FVT_lib/outp/OverrideAndLimit  SystemSampleTime=-1  VariantActivationTime=update diagram  Latency=0  AutoFrameSizeCalculation=off
      link override Signal_Limit/_maxval: Value=KOUTP_Awake_enum_maxval
      link override Signal_Limit/_minval: Value=KOUTP_Awake_enum_minval
      link override Signal_Override/_ovrdflg: Value=KOUTP_Awake_enum_ovrdflg
      link override Signal_Override/_ovrdval: Value=KOUTP_Awake_enum_ovrdval
  VNMM_CSB_flg_Inproc : FVT_lib/outp/OverrideAndLimit  SystemSampleTime=-1  VariantActivationTime=update diagram  Latency=0  AutoFrameSizeCalculation=off
      link override Signal_Limit/_maxval: Value=KOUTP_CSB_flg_maxval
      link override Signal_Limit/_minval: Value=KOUTP_CSB_flg_minval
      link override Signal_Override/_ovrdflg: Value=KOUTP_CSB_flg_ovrdflg
      link override Signal_Override/_ovrdval: Value=KOUTP_CSB_flg_ovrdval
  VNMM_ErrorState_enum_Inproc : FVT_lib/outp/OverrideAndLimit  SystemSampleTime=-1  VariantActivationTime=update diagram  Latency=0  AutoFrameSizeCalculation=off
      link override Signal_Limit/_maxval: Value=KOUTP_ErrorState_enum_maxval
      link override Signal_Limit/_minval: Value=KOUTP_ErrorState_enum_minval
      link override Signal_Override/_ovrdflg: Value=KOUTP_ErrorState_enum_ovrdflg
      link override Signal_Override/_ovrdval: Value=KOUTP_ErrorState_enum_ovrdval
  VNMM_NMmTxReq_flg_Inproc : FVT_lib/outp/OverrideAndLimit  SystemSampleTime=-1  VariantActivationTime=update diagram  Latency=0  AutoFrameSizeCalculation=off
      link override Signal_Limit/_maxval: Value=KOUTP_NMmTxReq_flg_maxval
      link override Signal_Limit/_minval: Value=KOUTP_NMmTxReq_flg_minval
      link override Signal_Override/_ovrdflg: Value=KOUTP_NMmTxReq_flg_ovrdflg
      link override Signal_Override/_ovrdval: Value=KOUTP_NMmTxReq_flg_ovrdval
  VNMM_NetworkReq_flg_Inproc : FVT_lib/outp/OverrideAndLimit  SystemSampleTime=-1  VariantActivationTime=update diagram  Latency=0  AutoFrameSizeCalculation=off
      link override Signal_Limit/_maxval: Value=KOUTP_NetworkReq_flg_maxval
      link override Signal_Limit/_minval: Value=KOUTP_NetworkReq_flg_minval
      link override Signal_Override/_ovrdflg: Value=KOUTP_NetworkReq_flg_ovrdflg
      link override Signal_Override/_ovrdval: Value=KOUTP_NetworkReq_flg_ovrdval
  VNMM_NodeID_enum_Inproc : FVT_lib/outp/OverrideAndLimit  SystemSampleTime=-1  VariantActivationTime=update diagram  Latency=0  AutoFrameSizeCalculation=off
      link override Signal_Limit/_maxval: Value=KOUTP_NodeID_enum_maxval
      link override Signal_Limit/_minval: Value=KOUTP_NodeID_enum_minval
      link override Signal_Override/_ovrdflg: Value=KOUTP_NodeID_enum_ovrdflg
      link override Signal_Override/_ovrdval: Value=KOUTP_NodeID_enum_ovrdval
  VNMM_PNI_flg_Inproc : FVT_lib/outp/OverrideAndLimit  SystemSampleTime=-1  VariantActivationTime=update diagram  Latency=0  AutoFrameSizeCalculation=off
      link override Signal_Limit/_maxval: Value=KOUTP_PNI_flg_maxval
      link override Signal_Limit/_minval: Value=KOUTP_PNI_flg_minval
      link override Signal_Override/_ovrdflg: Value=KOUTP_PNI_flg_ovrdflg
      link override Signal_Override/_ovrdval: Value=KOUTP_PNI_flg_ovrdval
  VNMM_RptMsgReq_flg_Inproc : FVT_lib/outp/OverrideAndLimit  SystemSampleTime=-1  VariantActivationTime=update diagram  Latency=0  AutoFrameSizeCalculation=off
      link override Signal_Limit/_maxval: Value=KOUTP_RptMsgReq_flg_maxval
      link override Signal_Limit/_minval: Value=KOUTP_RptMsgReq_flg_minval
      link override Signal_Override/_ovrdflg: Value=KOUTP_RptMsgReq_flg_ovrdflg
      link override Signal_Override/_ovrdval: Value=KOUTP_RptMsgReq_flg_ovrdval
  VNMM_SysNMmSta_enum_Inproc : FVT_lib/outp/OverrideAndLimit  SystemSampleTime=-1  VariantActivationTime=update diagram  Latency=0  AutoFrameSizeCalculation=off
      link override Signal_Limit/_maxval: Value=KOUTP_SysNMmSta_enum_maxval
      link override Signal_Limit/_minval: Value=KOUTP_SysNMmSta_enum_minval
      link override Signal_Override/_ovrdflg: Value=KOUTP_SysNMmSta_enum_ovrdflg
      link override Signal_Override/_ovrdval: Value=KOUTP_SysNMmSta_enum_ovrdval
  VNMM_WakeUp_enum_Inproc : FVT_lib/outp/OverrideAndLimit  SystemSampleTime=-1  VariantActivationTime=update diagram  Latency=0  AutoFrameSizeCalculation=off
      link override Signal_Limit/_maxval: Value=KOUTP_WakeUp_enum_maxval
      link override Signal_Limit/_minval: Value=KOUTP_WakeUp_enum_minval
      link override Signal_Override/_ovrdflg: Value=KOUTP_WakeUp_enum_ovrdflg
      link override Signal_Override/_ovrdval: Value=KOUTP_WakeUp_enum_ovrdval
  VPMM_ActiveDischargeReq_flg_Inproc : FVT_lib/outp/OverrideAndLimit  SystemSampleTime=-1  VariantActivationTime=update diagram  Latency=0  AutoFrameSizeCalculation=off
      link override Signal_Limit/_maxval: Value=KOUTP_ActiveDischargeReq_flg_maxval
      link override Signal_Limit/_minval: Value=KOUTP_ActiveDischargeReq_flg_minval
      link override Signal_Override/_ovrdflg: Value=KOUTP_ActiveDischargeReq_flg_ovrdflg
      link override Signal_Override/_ovrdval: Value=KOUTP_ActiveDischargeReq_flg_ovrdval
  VPMM_CtrlDrPwrStbA2_flg_Inproc : FVT_lib/outp/OverrideAndLimit  SystemSampleTime=-1  VariantActivationTime=update diagram  Latency=0  AutoFrameSizeCalculation=off
      link override Signal_Limit/_maxval: Value=KOUTP_CtrlDrPwrStbA2_flg_maxval
      link override Signal_Limit/_minval: Value=KOUTP_CtrlDrPwrStbA2_flg_minval
      link override Signal_Override/_ovrdflg: Value=KOUTP_CtrlDrPwrStbA2_flg_ovrdflg
      link override Signal_Override/_ovrdval: Value=KOUTP_CtrlDrPwrStbA2_flg_ovrdval
  VPMM_CtrlFrBMSCCUCIR_flg_Inproc : FVT_lib/outp/OverrideAndLimit  SystemSampleTime=-1  VariantActivationTime=update diagram  Latency=0  AutoFrameSizeCalculation=off
      link override Signal_Limit/_maxval: Value=KOUTP_CtrlFrBMSCCUCIR_flg_maxval
      link override Signal_Limit/_minval: Value=KOUTP_CtrlFrBMSCCUCIR_flg_minval
      link override Signal_Override/_ovrdflg: Value=KOUTP_CtrlFrBMSCCUCIR_flg_ovrdflg
      link override Signal_Override/_ovrdval: Value=KOUTP_CtrlFrBMSCCUCIR_flg_ovrdval
  VPMM_CtrlFrEDUINVERTER_flg_Inproc : FVT_lib/outp/OverrideAndLimit  SystemSampleTime=-1  VariantActivationTime=update diagram  Latency=0  AutoFrameSizeCalculation=off
      link override Signal_Limit/_maxval: Value=KOUTP_CtrlFrEDUINVERTER_flg_maxval
      link override Signal_Limit/_minval: Value=KOUTP_CtrlFrEDUINVERTER_flg_minval
      link override Signal_Override/_ovrdflg: Value=KOUTP_CtrlFrEDUINVERTER_flg_ovrdflg
      link override Signal_Override/_ovrdval: Value=KOUTP_CtrlFrEDUINVERTER_flg_ovrdval
  VPMM_CtrlFrPwrStbA1P_flg_Inproc : FVT_lib/outp/OverrideAndLimit  SystemSampleTime=-1  VariantActivationTime=update diagram  Latency=0  AutoFrameSizeCalculation=off
      link override Signal_Limit/_maxval: Value=KOUTP_CtrlFrPwrStbA1P_flg_maxval
      link override Signal_Limit/_minval: Value=KOUTP_CtrlFrPwrStbA1P_flg_minval
      link override Signal_Override/_ovrdflg: Value=KOUTP_CtrlFrPwrStbA1P_flg_ovrdflg
      link override Signal_Override/_ovrdval: Value=KOUTP_CtrlFrPwrStbA1P_flg_ovrdval
  VPMM_CtrlFrRC1_flg_Inproc : FVT_lib/outp/OverrideAndLimit  SystemSampleTime=-1  VariantActivationTime=update diagram  Latency=0  AutoFrameSizeCalculation=off
      link override Signal_Limit/_maxval: Value=KOUTP_CtrlFrRC1_flg_maxval
      link override Signal_Limit/_minval: Value=KOUTP_CtrlFrRC1_flg_minval
      link override Signal_Override/_ovrdflg: Value=KOUTP_CtrlFrRC1_flg_ovrdflg
      link override Signal_Override/_ovrdval: Value=KOUTP_CtrlFrRC1_flg_ovrdval
  VPMM_DCDCEnaReq_flg_Inproc : FVT_lib/outp/OverrideAndLimit  SystemSampleTime=-1  VariantActivationTime=update diagram  Latency=0  AutoFrameSizeCalculation=off
      link override Signal_Limit/_maxval: Value=KOUTP_DCDCEnaReq_flg_maxval
      link override Signal_Limit/_minval: Value=KOUTP_DCDCEnaReq_flg_minval
      link override Signal_Override/_ovrdflg: Value=KOUTP_DCDCEnaReq_flg_ovrdflg
      link override Signal_Override/_ovrdval: Value=KOUTP_DCDCEnaReq_flg_ovrdval
  VPMM_DCDCVoltSetpoint_V_Inproc : FVT_lib/outp/OverrideAndLimit  SystemSampleTime=-1  VariantActivationTime=update diagram  Latency=0  AutoFrameSizeCalculation=off
      link override Signal_Limit/_maxval: Value=KOUTP_DCDCVoltSetpoint_V_maxval
      link override Signal_Limit/_minval: Value=KOUTP_DCDCVoltSetpoint_V_minval
      link override Signal_Override/_ovrdflg: Value=KOUTP_DCDCVoltSetpoint_V_ovrdflg
      link override Signal_Override/_ovrdval: Value=KOUTP_DCDCVoltSetpoint_V_ovrdval
  VPMM_DrSeatSta_enum_Inproc : FVT_lib/outp/OverrideAndLimit  SystemSampleTime=-1  VariantActivationTime=update diagram  Latency=0  AutoFrameSizeCalculation=off
      link override Signal_Limit/_maxval: Value=KOUTP_DrSeatSta_enum_maxval
      link override Signal_Limit/_minval: Value=KOUTP_DrSeatSta_enum_minval
      link override Signal_Override/_ovrdflg: Value=KOUTP_DrSeatSta_enum_ovrdflg
      link override Signal_Override/_ovrdval: Value=KOUTP_DrSeatSta_enum_ovrdval
  VPMM_DrivetrainSelect_enum_Inproc : FVT_lib/outp/OverrideAndLimit  SystemSampleTime=-1  VariantActivationTime=update diagram  Latency=0  AutoFrameSizeCalculation=off
      link override Signal_Limit/_maxval: Value=KOUTP_DrivetrainSelect_enum_maxval
      link override Signal_Limit/_minval: Value=KOUTP_DrivetrainSelect_enum_minval
      link override Signal_Override/_ovrdflg: Value=KOUTP_DrivetrainSelect_enum_ovrdflg
      link override Signal_Override/_ovrdval: Value=KOUTP_DrivetrainSelect_enum_ovrdval
  VPMM_EvccAplusPwrUpReq_flg_Inproc : FVT_lib/outp/OverrideAndLimit  SystemSampleTime=-1  VariantActivationTime=update diagram  Latency=0  AutoFrameSizeCalculation=off
      link override Signal_Limit/_maxval: Value=KOUTP_EvccAplusPwrUpReq_flg_maxval
      link override Signal_Limit/_minval: Value=KOUTP_EvccAplusPwrUpReq_flg_minval
      link override Signal_Override/_ovrdflg: Value=KOUTP_EvccAplusPwrUpReq_flg_ovrdflg
      link override Signal_Override/_ovrdval: Value=KOUTP_EvccAplusPwrUpReq_flg_ovrdval
  VPMM_FDADC12VDetAvg_mV_Inproc : FVT_lib/outp/OverrideAndLimit  SystemSampleTime=-1  VariantActivationTime=update diagram  Latency=0  AutoFrameSizeCalculation=off
      link override Signal_Limit/_maxval: Value=KOUTP_FDADC12VDetAvg_mV_maxval
      link override Signal_Limit/_minval: Value=KOUTP_FDADC12VDetAvg_mV_minval
      link override Signal_Override/_ovrdflg: Value=KOUTP_FDADC12VDetAvg_mV_ovrdflg
      link override Signal_Override/_ovrdval: Value=KOUTP_FDADC12VDetAvg_mV_ovrdval
  VPMM_FrMCUEnaReq_flg_Inproc : FVT_lib/outp/OverrideAndLimit  SystemSampleTime=-1  VariantActivationTime=update diagram  Latency=0  AutoFrameSizeCalculation=off
      link override Signal_Limit/_maxval: Value=KOUTP_FrMCUEnaReq_flg_maxval
      link override Signal_Limit/_minval: Value=KOUTP_FrMCUEnaReq_flg_minval
      link override Signal_Override/_ovrdflg: Value=KOUTP_FrMCUEnaReq_flg_ovrdflg
      link override Signal_Override/_ovrdval: Value=KOUTP_FrMCUEnaReq_flg_ovrdval
  VPMM_HVBatCnctReq_flg_Inproc : FVT_lib/outp/OverrideAndLimit  SystemSampleTime=-1  VariantActivationTime=update diagram  Latency=0  AutoFrameSizeCalculation=off
      link override Signal_Limit/_maxval: Value=KOUTP_HVBatCnctReq_flg_maxval
      link override Signal_Limit/_minval: Value=KOUTP_HVBatCnctReq_flg_minval
      link override Signal_Override/_ovrdflg: Value=KOUTP_HVBatCnctReq_flg_ovrdflg
      link override Signal_Override/_ovrdval: Value=KOUTP_HVBatCnctReq_flg_ovrdval
  VPMM_HVPwrSta_flg_Inproc : FVT_lib/outp/OverrideAndLimit  SystemSampleTime=-1  VariantActivationTime=update diagram  Latency=0  AutoFrameSizeCalculation=off
      link override Signal_Limit/_maxval: Value=KOUTP_HVPwrSta_flg_maxval
      link override Signal_Limit/_minval: Value=KOUTP_HVPwrSta_flg_minval
      link override Signal_Override/_ovrdflg: Value=KOUTP_HVPwrSta_flg_ovrdflg
      link override Signal_Override/_ovrdval: Value=KOUTP_HVPwrSta_flg_ovrdval
  VPMM_HVSysReadyToCharge_enum_Inproc : FVT_lib/outp/OverrideAndLimit  SystemSampleTime=-1  VariantActivationTime=update diagram  Latency=0  AutoFrameSizeCalculation=off
      link override Signal_Limit/_maxval: Value=KOUTP_HVSysReadyToCharge_enum_maxval
      link override Signal_Limit/_minval: Value=KOUTP_HVSysReadyToCharge_enum_minval
      link override Signal_Override/_ovrdflg: Value=KOUTP_HVSysReadyToCharge_enum_ovrdflg
      link override Signal_Override/_ovrdval: Value=KOUTP_HVSysReadyToCharge_enum_ovrdval
  VPMM_HWResetSta_enum_Inproc : FVT_lib/outp/OverrideAndLimit  SystemSampleTime=-1  VariantActivationTime=update diagram  Latency=0  AutoFrameSizeCalculation=off
      link override Signal_Limit/_maxval: Value=KOUTP_HWResetSta_enum_maxval
      link override Signal_Limit/_minval: Value=KOUTP_HWResetSta_enum_minval
      link override Signal_Override/_ovrdflg: Value=KOUTP_HWResetSta_enum_ovrdflg
      link override Signal_Override/_ovrdval: Value=KOUTP_HWResetSta_enum_ovrdval
  VPMM_IVIPwrStaONTOPopT_s_Inproc : FVT_lib/outp/OverrideAndLimit  SystemSampleTime=-1  VariantActivationTime=update diagram  Latency=0  AutoFrameSizeCalculation=off
      link override Signal_Limit/_maxval: Value=KOUTP_IVIPwrStaONTOPopT_s_maxval
      link override Signal_Limit/_minval: Value=KOUTP_IVIPwrStaONTOPopT_s_minval
      link override Signal_Override/_ovrdflg: Value=KOUTP_IVIPwrStaONTOPopT_s_ovrdflg
      link override Signal_Override/_ovrdval: Value=KOUTP_IVIPwrStaONTOPopT_s_ovrdval
  VPMM_LVBattChrgTimeCnt_s_Inproc : FVT_lib/outp/OverrideAndLimit  SystemSampleTime=-1  VariantActivationTime=update diagram  Latency=0  AutoFrameSizeCalculation=off
      link override Signal_Limit/_maxval: Value=KOUTP_LVBattChrgTimeCnt_s_maxval
      link override Signal_Limit/_minval: Value=KOUTP_LVBattChrgTimeCnt_s_minval
      link override Signal_Override/_ovrdflg: Value=KOUTP_LVBattChrgTimeCnt_s_ovrdflg
      link override Signal_Override/_ovrdval: Value=KOUTP_LVBattChrgTimeCnt_s_ovrdval
  VPMM_LVChrgHoldTtimer_s_Inproc : FVT_lib/outp/OverrideAndLimit  SystemSampleTime=-1  VariantActivationTime=update diagram  Latency=0  AutoFrameSizeCalculation=off
      link override Signal_Limit/_maxval: Value=KOUTP_LVChrgHoldTtimer_s_maxval
      link override Signal_Limit/_minval: Value=KOUTP_LVChrgHoldTtimer_s_minval
      link override Signal_Override/_ovrdflg: Value=KOUTP_LVChrgHoldTtimer_s_ovrdflg
      link override Signal_Override/_ovrdval: Value=KOUTP_LVChrgHoldTtimer_s_ovrdval
  VPMM_LVPwrSta_flg_Inproc : FVT_lib/outp/OverrideAndLimit  SystemSampleTime=-1  VariantActivationTime=update diagram  Latency=0  AutoFrameSizeCalculation=off
      link override Signal_Limit/_maxval: Value=KOUTP_LVPwrSta_flg_maxval
      link override Signal_Limit/_minval: Value=KOUTP_LVPwrSta_flg_minval
      link override Signal_Override/_ovrdflg: Value=KOUTP_LVPwrSta_flg_ovrdflg
      link override Signal_Override/_ovrdval: Value=KOUTP_LVPwrSta_flg_ovrdval
  VPMM_LVSilentChrgLv_enum_Inproc : FVT_lib/outp/OverrideAndLimit  SystemSampleTime=-1  VariantActivationTime=update diagram  Latency=0  AutoFrameSizeCalculation=off
      link override Signal_Limit/_maxval: Value=KOUTP_LVSilentChrgLv_enum_maxval
      link override Signal_Limit/_minval: Value=KOUTP_LVSilentChrgLv_enum_minval
      link override Signal_Override/_ovrdflg: Value=KOUTP_LVSilentChrgLv_enum_ovrdflg
      link override Signal_Override/_ovrdval: Value=KOUTP_LVSilentChrgLv_enum_ovrdval
  VPMM_LVSilentChrgReq_flg_Inproc : FVT_lib/outp/OverrideAndLimit  SystemSampleTime=-1  VariantActivationTime=update diagram  Latency=0  AutoFrameSizeCalculation=off
      link override Signal_Limit/_maxval: Value=KOUTP_LVSilentChrgReq_flg_maxval
      link override Signal_Limit/_minval: Value=KOUTP_LVSilentChrgReq_flg_minval
      link override Signal_Override/_ovrdflg: Value=KOUTP_LVSilentChrgReq_flg_ovrdflg
      link override Signal_Override/_ovrdval: Value=KOUTP_LVSilentChrgReq_flg_ovrdval
  VPMM_LVSilentChrgSta_enum_Inproc : FVT_lib/outp/OverrideAndLimit  SystemSampleTime=-1  VariantActivationTime=update diagram  Latency=0  AutoFrameSizeCalculation=off
      link override Signal_Limit/_maxval: Value=KOUTP_LVSilentChrgSta_enum_maxval
      link override Signal_Limit/_minval: Value=KOUTP_LVSilentChrgSta_enum_minval
      link override Signal_Override/_ovrdflg: Value=KOUTP_LVSilentChrgSta_enum_ovrdflg
      link override Signal_Override/_ovrdval: Value=KOUTP_LVSilentChrgSta_enum_ovrdval
  VPMM_LowSOCWarn_enum_Inproc : FVT_lib/outp/OverrideAndLimit  SystemSampleTime=-1  VariantActivationTime=update diagram  Latency=0  AutoFrameSizeCalculation=off
      link override Signal_Limit/_maxval: Value=KOUTP_LowSOCWarn_enum_maxval
      link override Signal_Limit/_minval: Value=KOUTP_LowSOCWarn_enum_minval
      link override Signal_Override/_ovrdflg: Value=KOUTP_LowSOCWarn_enum_ovrdflg
      link override Signal_Override/_ovrdval: Value=KOUTP_LowSOCWarn_enum_ovrdval
  VPMM_OTAPwrReqOFFChkSta_enum_Inproc : FVT_lib/outp/OverrideAndLimit  SystemSampleTime=-1  VariantActivationTime=update diagram  Latency=0  AutoFrameSizeCalculation=off
      link override Signal_Limit/_maxval: Value=KOUTP_OTAPwrReqOFFChkSta_enum_maxval
      link override Signal_Limit/_minval: Value=KOUTP_OTAPwrReqOFFChkSta_enum_minval
      link override Signal_Override/_ovrdflg: Value=KOUTP_OTAPwrReqOFFChkSta_enum_ovrdflg
      link override Signal_Override/_ovrdval: Value=KOUTP_OTAPwrReqOFFChkSta_enum_ovrdval
  VPMM_OTAPwrReqStdChkSta_enum_Inproc : FVT_lib/outp/OverrideAndLimit  SystemSampleTime=-1  VariantActivationTime=update diagram  Latency=0  AutoFrameSizeCalculation=off
      link override Signal_Limit/_maxval: Value=KOUTP_OTAPwrReqStdChkSta_enum_maxval
      link override Signal_Limit/_minval: Value=KOUTP_OTAPwrReqStdChkSta_enum_minval
      link override Signal_Override/_ovrdflg: Value=KOUTP_OTAPwrReqStdChkSta_enum_ovrdflg
      link override Signal_Override/_ovrdval: Value=KOUTP_OTAPwrReqStdChkSta_enum_ovrdval
  VPMM_PMMAllowECUSleep_flg_Inproc : FVT_lib/outp/OverrideAndLimit  SystemSampleTime=-1  VariantActivationTime=update diagram  Latency=0  AutoFrameSizeCalculation=off
      link override Signal_Limit/_maxval: Value=KOUTP_PMMAllowECUSleep_flg_maxval
      link override Signal_Limit/_minval: Value=KOUTP_PMMAllowECUSleep_flg_minval
      link override Signal_Override/_ovrdflg: Value=KOUTP_PMMAllowECUSleep_flg_ovrdflg
      link override Signal_Override/_ovrdval: Value=KOUTP_PMMAllowECUSleep_flg_ovrdval
  VPMM_PowerDownFault_enum_Inproc : FVT_lib/outp/OverrideAndLimit  SystemSampleTime=-1  VariantActivationTime=update diagram  Latency=0  AutoFrameSizeCalculation=off
      link override Signal_Limit/_maxval: Value=KOUTP_PowerDownFault_enum_maxval
      link override Signal_Limit/_minval: Value=KOUTP_PowerDownFault_enum_minval
      link override Signal_Override/_ovrdflg: Value=KOUTP_PowerDownFault_enum_ovrdflg
      link override Signal_Override/_ovrdval: Value=KOUTP_PowerDownFault_enum_ovrdval
  VPMM_PowerDownState_enum_Inproc : FVT_lib/outp/OverrideAndLimit  SystemSampleTime=-1  VariantActivationTime=update diagram  Latency=0  AutoFrameSizeCalculation=off
      link override Signal_Limit/_maxval: Value=KOUTP_PowerDownState_enum_maxval
      link override Signal_Limit/_minval: Value=KOUTP_PowerDownState_enum_minval
      link override Signal_Override/_ovrdflg: Value=KOUTP_PowerDownState_enum_ovrdflg
      link override Signal_Override/_ovrdval: Value=KOUTP_PowerDownState_enum_ovrdval
  VPMM_PowerSta_enum_Inproc : FVT_lib/outp/OverrideAndLimit  SystemSampleTime=-1  VariantActivationTime=update diagram  Latency=0  AutoFrameSizeCalculation=off
      link override Signal_Limit/_maxval: Value=KOUTP_PowerSta_enum_maxval
      link override Signal_Limit/_minval: Value=KOUTP_PowerSta_enum_minval
      link override Signal_Override/_ovrdflg: Value=KOUTP_PowerSta_enum_ovrdflg
      link override Signal_Override/_ovrdval: Value=KOUTP_PowerSta_enum_ovrdval
  VPMM_PowerUpFault_enum_Inproc : FVT_lib/outp/OverrideAndLimit  SystemSampleTime=-1  VariantActivationTime=update diagram  Latency=0  AutoFrameSizeCalculation=off
      link override Signal_Limit/_maxval: Value=KOUTP_PowerUpFault_enum_maxval
      link override Signal_Limit/_minval: Value=KOUTP_PowerUpFault_enum_minval
      link override Signal_Override/_ovrdflg: Value=KOUTP_PowerUpFault_enum_ovrdflg
      link override Signal_Override/_ovrdval: Value=KOUTP_PowerUpFault_enum_ovrdval
  VPMM_PowerUpState_enum_Inproc : FVT_lib/outp/OverrideAndLimit  SystemSampleTime=-1  VariantActivationTime=update diagram  Latency=0  AutoFrameSizeCalculation=off
      link override Signal_Limit/_maxval: Value=KOUTP_PowerUpState_enum_maxval
      link override Signal_Limit/_minval: Value=KOUTP_PowerUpState_enum_minval
      link override Signal_Override/_ovrdflg: Value=KOUTP_PowerUpState_enum_ovrdflg
      link override Signal_Override/_ovrdval: Value=KOUTP_PowerUpState_enum_ovrdval
  VPMM_PwrDownReq_enum_Inproc : FVT_lib/outp/OverrideAndLimit  SystemSampleTime=-1  VariantActivationTime=update diagram  Latency=0  AutoFrameSizeCalculation=off
      link override Signal_Limit/_maxval: Value=KOUTP_PwrDownReq_enum_maxval
      link override Signal_Limit/_minval: Value=KOUTP_PwrDownReq_enum_minval
      link override Signal_Override/_ovrdflg: Value=KOUTP_PwrDownReq_enum_ovrdflg
      link override Signal_Override/_ovrdval: Value=KOUTP_PwrDownReq_enum_ovrdval
  VPMM_PwrReqRAPSAvail_flg_Inproc : FVT_lib/outp/OverrideAndLimit  SystemSampleTime=-1  VariantActivationTime=update diagram  Latency=0  AutoFrameSizeCalculation=off
      link override Signal_Limit/_maxval: Value=KOUTP_PwrReqRAPSAvail_flg_maxval
      link override Signal_Limit/_minval: Value=KOUTP_PwrReqRAPSAvail_flg_minval
      link override Signal_Override/_ovrdflg: Value=KOUTP_PwrReqRAPSAvail_flg_ovrdflg
      link override Signal_Override/_ovrdval: Value=KOUTP_PwrReqRAPSAvail_flg_ovrdval
  VPMM_PwrReq_OTA_enum_Inproc : FVT_lib/outp/OverrideAndLimit  SystemSampleTime=-1  VariantActivationTime=update diagram  Latency=0  AutoFrameSizeCalculation=off
      link override Signal_Limit/_maxval: Value=KOUTP_PwrReq_OTA_enum_maxval
      link override Signal_Limit/_minval: Value=KOUTP_PwrReq_OTA_enum_minval
      link override Signal_Override/_ovrdflg: Value=KOUTP_PwrReq_OTA_enum_ovrdflg
      link override Signal_Override/_ovrdval: Value=KOUTP_PwrReq_OTA_enum_ovrdval
  VPMM_PwrStaConstraint_enum_Inproc : FVT_lib/outp/OverrideAndLimit  SystemSampleTime=-1  VariantActivationTime=update diagram  Latency=0  AutoFrameSizeCalculation=off
      link override Signal_Limit/_maxval: Value=KOUTP_PwrStaConstraint_enum_maxval
      link override Signal_Limit/_minval: Value=KOUTP_PwrStaConstraint_enum_minval
      link override Signal_Override/_ovrdflg: Value=KOUTP_PwrStaConstraint_enum_ovrdflg
      link override Signal_Override/_ovrdval: Value=KOUTP_PwrStaConstraint_enum_ovrdval
  VPMM_PwrStaONTOPopReq_flg_Inproc : FVT_lib/outp/OverrideAndLimit  SystemSampleTime=-1  VariantActivationTime=update diagram  Latency=0  AutoFrameSizeCalculation=off
      link override Signal_Limit/_maxval: Value=KOUTP_PwrStaONTOPopReq_flg_maxval
      link override Signal_Limit/_minval: Value=KOUTP_PwrStaONTOPopReq_flg_minval
      link override Signal_Override/_ovrdflg: Value=KOUTP_PwrStaONTOPopReq_flg_ovrdflg
      link override Signal_Override/_ovrdval: Value=KOUTP_PwrStaONTOPopReq_flg_ovrdval
  VPMM_PwrStaSelect_enum_Inproc : FVT_lib/outp/OverrideAndLimit  SystemSampleTime=-1  VariantActivationTime=update diagram  Latency=0  AutoFrameSizeCalculation=off
      link override Signal_Limit/_maxval: Value=KOUTP_PwrStaSelect_enum_maxval
      link override Signal_Limit/_minval: Value=KOUTP_PwrStaSelect_enum_minval
      link override Signal_Override/_ovrdflg: Value=KOUTP_PwrStaSelect_enum_ovrdflg
      link override Signal_Override/_ovrdval: Value=KOUTP_PwrStaSelect_enum_ovrdval
  VPMM_PwrStaTOSta_enum_Inproc : FVT_lib/outp/OverrideAndLimit  SystemSampleTime=-1  VariantActivationTime=update diagram  Latency=0  AutoFrameSizeCalculation=off
      link override Signal_Limit/_maxval: Value=KOUTP_PwrStaTOSta_enum_maxval
      link override Signal_Limit/_minval: Value=KOUTP_PwrStaTOSta_enum_minval
      link override Signal_Override/_ovrdflg: Value=KOUTP_PwrStaTOSta_enum_ovrdflg
      link override Signal_Override/_ovrdval: Value=KOUTP_PwrStaTOSta_enum_ovrdval
  VPMM_PwrUpReq_enum_Inproc : FVT_lib/outp/OverrideAndLimit  SystemSampleTime=-1  VariantActivationTime=update diagram  Latency=0  AutoFrameSizeCalculation=off
      link override Signal_Limit/_maxval: Value=KOUTP_PwrUpReq_enum_maxval
      link override Signal_Limit/_minval: Value=KOUTP_PwrUpReq_enum_minval
      link override Signal_Override/_ovrdflg: Value=KOUTP_PwrUpReq_enum_ovrdflg
      link override Signal_Override/_ovrdval: Value=KOUTP_PwrUpReq_enum_ovrdval
  VPMM_ReVehThdChkSta_enum_Inproc : FVT_lib/outp/OverrideAndLimit  SystemSampleTime=-1  VariantActivationTime=update diagram  Latency=0  AutoFrameSizeCalculation=off
      link override Signal_Limit/_maxval: Value=KOUTP_ReVehThdChkSta_enum_maxval
      link override Signal_Limit/_minval: Value=KOUTP_ReVehThdChkSta_enum_minval
      link override Signal_Override/_ovrdflg: Value=KOUTP_ReVehThdChkSta_enum_ovrdflg
      link override Signal_Override/_ovrdval: Value=KOUTP_ReVehThdChkSta_enum_ovrdval
  VPMM_RrMCUEnaReq_flg_Inproc : FVT_lib/outp/OverrideAndLimit  SystemSampleTime=-1  VariantActivationTime=update diagram  Latency=0  AutoFrameSizeCalculation=off
      link override Signal_Limit/_maxval: Value=KOUTP_RrMCUEnaReq_flg_maxval
      link override Signal_Limit/_minval: Value=KOUTP_RrMCUEnaReq_flg_minval
      link override Signal_Override/_ovrdflg: Value=KOUTP_RrMCUEnaReq_flg_ovrdflg
      link override Signal_Override/_ovrdval: Value=KOUTP_RrMCUEnaReq_flg_ovrdval
  VPMM_Sched_ChgTOSta_enum_Inproc : FVT_lib/outp/OverrideAndLimit  SystemSampleTime=-1  VariantActivationTime=update diagram  Latency=0  AutoFrameSizeCalculation=off
      link override Signal_Limit/_maxval: Value=KOUTP_Sched_ChgTOSta_enum_maxval
      link override Signal_Limit/_minval: Value=KOUTP_Sched_ChgTOSta_enum_minval
      link override Signal_Override/_ovrdflg: Value=KOUTP_Sched_ChgTOSta_enum_ovrdflg
      link override Signal_Override/_ovrdval: Value=KOUTP_Sched_ChgTOSta_enum_ovrdval
  VPMM_SilentChkAllowSleep_flg_Inproc : FVT_lib/outp/OverrideAndLimit  SystemSampleTime=-1  VariantActivationTime=update diagram  Latency=0  AutoFrameSizeCalculation=off
      link override Signal_Limit/_maxval: Value=KOUTP_SilentChkAllowSleep_flg_maxval
      link override Signal_Limit/_minval: Value=KOUTP_SilentChkAllowSleep_flg_minval
      link override Signal_Override/_ovrdflg: Value=KOUTP_SilentChkAllowSleep_flg_ovrdflg
      link override Signal_Override/_ovrdval: Value=KOUTP_SilentChkAllowSleep_flg_ovrdval
  VPMM_SysPowerMode_enum_Inproc : FVT_lib/outp/OverrideAndLimit  SystemSampleTime=-1  VariantActivationTime=update diagram  Latency=0  AutoFrameSizeCalculation=off
      link override Signal_Limit/_maxval: Value=KOUTP_SysPowerMode_enum_maxval
      link override Signal_Limit/_minval: Value=KOUTP_SysPowerMode_enum_minval
      link override Signal_Override/_ovrdflg: Value=KOUTP_SysPowerMode_enum_ovrdflg
      link override Signal_Override/_ovrdval: Value=KOUTP_SysPowerMode_enum_ovrdval
  VPMM_TCountSta_enum_Inproc : FVT_lib/outp/OverrideAndLimit  SystemSampleTime=-1  VariantActivationTime=update diagram  Latency=0  AutoFrameSizeCalculation=off
      link override Signal_Limit/_maxval: Value=KOUTP_TCountSta_enum_maxval
      link override Signal_Limit/_minval: Value=KOUTP_TCountSta_enum_minval
      link override Signal_Override/_ovrdflg: Value=KOUTP_TCountSta_enum_ovrdflg
      link override Signal_Override/_ovrdval: Value=KOUTP_TCountSta_enum_ovrdval
  VPMM_TimerAllowSleep_flg_Inproc : FVT_lib/outp/OverrideAndLimit  SystemSampleTime=-1  VariantActivationTime=update diagram  Latency=0  AutoFrameSizeCalculation=off
      link override Signal_Limit/_maxval: Value=KOUTP_TimerAllowSleep_flg_maxval
      link override Signal_Limit/_minval: Value=KOUTP_TimerAllowSleep_flg_minval
      link override Signal_Override/_ovrdflg: Value=KOUTP_TimerAllowSleep_flg_ovrdflg
      link override Signal_Override/_ovrdval: Value=KOUTP_TimerAllowSleep_flg_ovrdval
  VSYS_AcoreRebootCmdACK_flg_Inproc : FVT_lib/outp/OverrideAndLimit  SystemSampleTime=-1  VariantActivationTime=update diagram  Latency=0  AutoFrameSizeCalculation=off
      link override Signal_Limit/_maxval: Value=KOUTP_AcoreRebootCmdACK_flg_maxval
      link override Signal_Limit/_minval: Value=KOUTP_AcoreRebootCmdACK_flg_minval
      link override Signal_Override/_ovrdflg: Value=KOUTP_AcoreRebootCmdACK_flg_ovrdflg
      link override Signal_Override/_ovrdval: Value=KOUTP_AcoreRebootCmdACK_flg_ovrdval
  VSYS_CarModel1_cnt_Inproc : FVT_lib/outp/OverrideAndLimit  SystemSampleTime=-1  VariantActivationTime=update diagram  Latency=0  AutoFrameSizeCalculation=off
      link override Signal_Limit/_maxval: Value=KOUTP_CarModel1_cnt_maxval
      link override Signal_Limit/_minval: Value=KOUTP_CarModel1_cnt_minval
      link override Signal_Override/_ovrdflg: Value=KOUTP_CarModel1_cnt_ovrdflg
      link override Signal_Override/_ovrdval: Value=KOUTP_CarModel1_cnt_ovrdval
  VSYS_CarModel2_cnt_Inproc : FVT_lib/outp/OverrideAndLimit  SystemSampleTime=-1  VariantActivationTime=update diagram  Latency=0  AutoFrameSizeCalculation=off
      link override Signal_Limit/_maxval: Value=KOUTP_CarModel2_cnt_maxval
      link override Signal_Limit/_minval: Value=KOUTP_CarModel2_cnt_minval
      link override Signal_Override/_ovrdflg: Value=KOUTP_CarModel2_cnt_ovrdflg
      link override Signal_Override/_ovrdval: Value=KOUTP_CarModel2_cnt_ovrdval
  VSYS_CarModel3_cnt_Inproc : FVT_lib/outp/OverrideAndLimit  SystemSampleTime=-1  VariantActivationTime=update diagram  Latency=0  AutoFrameSizeCalculation=off
      link override Signal_Limit/_maxval: Value=KOUTP_CarModel3_cnt_maxval
      link override Signal_Limit/_minval: Value=KOUTP_CarModel3_cnt_minval
      link override Signal_Override/_ovrdflg: Value=KOUTP_CarModel3_cnt_ovrdflg
      link override Signal_Override/_ovrdval: Value=KOUTP_CarModel3_cnt_ovrdval
  VSYS_Change1_cnt_Inproc : FVT_lib/outp/OverrideAndLimit  SystemSampleTime=-1  VariantActivationTime=update diagram  Latency=0  AutoFrameSizeCalculation=off
      link override Signal_Limit/_maxval: Value=KOUTP_Change1_cnt_maxval
      link override Signal_Limit/_minval: Value=KOUTP_Change1_cnt_minval
      link override Signal_Override/_ovrdflg: Value=KOUTP_Change1_cnt_ovrdflg
      link override Signal_Override/_ovrdval: Value=KOUTP_Change1_cnt_ovrdval
  VSYS_Change2_cnt_Inproc : FVT_lib/outp/OverrideAndLimit  SystemSampleTime=-1  VariantActivationTime=update diagram  Latency=0  AutoFrameSizeCalculation=off
      link override Signal_Limit/_maxval: Value=KOUTP_Change2_cnt_maxval
      link override Signal_Limit/_minval: Value=KOUTP_Change2_cnt_minval
      link override Signal_Override/_ovrdflg: Value=KOUTP_Change2_cnt_ovrdflg
      link override Signal_Override/_ovrdval: Value=KOUTP_Change2_cnt_ovrdval
  VSYS_Country1_cnt_Inproc : FVT_lib/outp/OverrideAndLimit  SystemSampleTime=-1  VariantActivationTime=update diagram  Latency=0  AutoFrameSizeCalculation=off
      link override Signal_Limit/_maxval: Value=KOUTP_Country1_cnt_maxval
      link override Signal_Limit/_minval: Value=KOUTP_Country1_cnt_minval
      link override Signal_Override/_ovrdflg: Value=KOUTP_Country1_cnt_ovrdflg
      link override Signal_Override/_ovrdval: Value=KOUTP_Country1_cnt_ovrdval
  VSYS_Country2_cnt_Inproc : FVT_lib/outp/OverrideAndLimit  SystemSampleTime=-1  VariantActivationTime=update diagram  Latency=0  AutoFrameSizeCalculation=off
      link override Signal_Limit/_maxval: Value=KOUTP_Country2_cnt_maxval
      link override Signal_Limit/_minval: Value=KOUTP_Country2_cnt_minval
      link override Signal_Override/_ovrdflg: Value=KOUTP_Country2_cnt_ovrdflg
      link override Signal_Override/_ovrdval: Value=KOUTP_Country2_cnt_ovrdval
  VSYS_CurrentNmState_enum_Inproc : FVT_lib/outp/OverrideAndLimit  SystemSampleTime=-1  VariantActivationTime=update diagram  Latency=0  AutoFrameSizeCalculation=off
      link override Signal_Limit/_maxval: Value=KOUTP_CurrentNmState_enum_maxval
      link override Signal_Limit/_minval: Value=KOUTP_CurrentNmState_enum_minval
      link override Signal_Override/_ovrdflg: Value=KOUTP_CurrentNmState_enum_ovrdflg
      link override Signal_Override/_ovrdval: Value=KOUTP_CurrentNmState_enum_ovrdval
  VSYS_Dash1_cnt_Inproc : FVT_lib/outp/OverrideAndLimit  SystemSampleTime=-1  VariantActivationTime=update diagram  Latency=0  AutoFrameSizeCalculation=off
      link override Signal_Limit/_maxval: Value=KOUTP_Dash1_cnt_maxval
      link override Signal_Limit/_minval: Value=KOUTP_Dash1_cnt_minval
      link override Signal_Override/_ovrdflg: Value=KOUTP_Dash1_cnt_ovrdflg
      link override Signal_Override/_ovrdval: Value=KOUTP_Dash1_cnt_ovrdval
  VSYS_Dash2_cnt_Inproc : FVT_lib/outp/OverrideAndLimit  SystemSampleTime=-1  VariantActivationTime=update diagram  Latency=0  AutoFrameSizeCalculation=off
      link override Signal_Limit/_maxval: Value=KOUTP_Dash2_cnt_maxval
      link override Signal_Limit/_minval: Value=KOUTP_Dash2_cnt_minval
      link override Signal_Override/_ovrdflg: Value=KOUTP_Dash2_cnt_ovrdflg
      link override Signal_Override/_ovrdval: Value=KOUTP_Dash2_cnt_ovrdval
  VSYS_DrivingMode_cnt_Inproc : FVT_lib/outp/OverrideAndLimit  SystemSampleTime=-1  VariantActivationTime=update diagram  Latency=0  AutoFrameSizeCalculation=off
      link override Signal_Limit/_maxval: Value=KOUTP_DrivingMode_cnt_maxval
      link override Signal_Limit/_minval: Value=KOUTP_DrivingMode_cnt_minval
      link override Signal_Override/_ovrdflg: Value=KOUTP_DrivingMode_cnt_ovrdflg
      link override Signal_Override/_ovrdval: Value=KOUTP_DrivingMode_cnt_ovrdval
  VSYS_ECU1_cnt_Inproc : FVT_lib/outp/OverrideAndLimit  SystemSampleTime=-1  VariantActivationTime=update diagram  Latency=0  AutoFrameSizeCalculation=off
      link override Signal_Limit/_maxval: Value=KOUTP_ECU1_cnt_maxval
      link override Signal_Limit/_minval: Value=KOUTP_ECU1_cnt_minval
      link override Signal_Override/_ovrdflg: Value=KOUTP_ECU1_cnt_ovrdflg
      link override Signal_Override/_ovrdval: Value=KOUTP_ECU1_cnt_ovrdval
  VSYS_ECU2_cnt_Inproc : FVT_lib/outp/OverrideAndLimit  SystemSampleTime=-1  VariantActivationTime=update diagram  Latency=0  AutoFrameSizeCalculation=off
      link override Signal_Limit/_maxval: Value=KOUTP_ECU2_cnt_maxval
      link override Signal_Limit/_minval: Value=KOUTP_ECU2_cnt_minval
      link override Signal_Override/_ovrdflg: Value=KOUTP_ECU2_cnt_ovrdflg
      link override Signal_Override/_ovrdval: Value=KOUTP_ECU2_cnt_ovrdval
  VSYS_ECUGen1_cnt_Inproc : FVT_lib/outp/OverrideAndLimit  SystemSampleTime=-1  VariantActivationTime=update diagram  Latency=0  AutoFrameSizeCalculation=off
      link override Signal_Limit/_maxval: Value=KOUTP_ECUGen1_cnt_maxval
      link override Signal_Limit/_minval: Value=KOUTP_ECUGen1_cnt_minval
      link override Signal_Override/_ovrdflg: Value=KOUTP_ECUGen1_cnt_ovrdflg
      link override Signal_Override/_ovrdval: Value=KOUTP_ECUGen1_cnt_ovrdval
  VSYS_ECUGen2_cnt_Inproc : FVT_lib/outp/OverrideAndLimit  SystemSampleTime=-1  VariantActivationTime=update diagram  Latency=0  AutoFrameSizeCalculation=off
      link override Signal_Limit/_maxval: Value=KOUTP_ECUGen2_cnt_maxval
      link override Signal_Limit/_minval: Value=KOUTP_ECUGen2_cnt_minval
      link override Signal_Override/_ovrdflg: Value=KOUTP_ECUGen2_cnt_ovrdflg
      link override Signal_Override/_ovrdval: Value=KOUTP_ECUGen2_cnt_ovrdval
  VSYS_FdcSlpReqRisingEdge_flg_Inproc : FVT_lib/outp/OverrideAndLimit  SystemSampleTime=-1  VariantActivationTime=update diagram  Latency=0  AutoFrameSizeCalculation=off
      link override Signal_Limit/_maxval: Value=KOUTP_FdcSlpReqRisingEdge_flg_maxval
      link override Signal_Limit/_minval: Value=KOUTP_FdcSlpReqRisingEdge_flg_minval
      link override Signal_Override/_ovrdflg: Value=KOUTP_FdcSlpReqRisingEdge_flg_ovrdflg
      link override Signal_Override/_ovrdval: Value=KOUTP_FdcSlpReqRisingEdge_flg_ovrdval
  VSYS_FdcSlpTime_sec_Inproc : FVT_lib/outp/OverrideAndLimit  SystemSampleTime=-1  VariantActivationTime=update diagram  Latency=0  AutoFrameSizeCalculation=off
      link override Signal_Limit/_maxval: Value=KOUTP_FdcSlpTime_sec_maxval
      link override Signal_Limit/_minval: Value=KOUTP_FdcSlpTime_sec_minval
      link override Signal_Override/_ovrdflg: Value=KOUTP_FdcSlpTime_sec_ovrdflg
      link override Signal_Override/_ovrdval: Value=KOUTP_FdcSlpTime_sec_ovrdval
  VSYS_HWVer1_cnt_Inproc : FVT_lib/outp/OverrideAndLimit  SystemSampleTime=-1  VariantActivationTime=update diagram  Latency=0  AutoFrameSizeCalculation=off
      link override Signal_Limit/_maxval: Value=KOUTP_HWVer1_cnt_maxval
      link override Signal_Limit/_minval: Value=KOUTP_HWVer1_cnt_minval
      link override Signal_Override/_ovrdflg: Value=KOUTP_HWVer1_cnt_ovrdflg
      link override Signal_Override/_ovrdval: Value=KOUTP_HWVer1_cnt_ovrdval
  VSYS_HWVer2_cnt_Inproc : FVT_lib/outp/OverrideAndLimit  SystemSampleTime=-1  VariantActivationTime=update diagram  Latency=0  AutoFrameSizeCalculation=off
      link override Signal_Limit/_maxval: Value=KOUTP_HWVer2_cnt_maxval
      link override Signal_Limit/_minval: Value=KOUTP_HWVer2_cnt_minval
      link override Signal_Override/_ovrdflg: Value=KOUTP_HWVer2_cnt_ovrdflg
      link override Signal_Override/_ovrdval: Value=KOUTP_HWVer2_cnt_ovrdval
  VSYS_HWVer3_cnt_Inproc : FVT_lib/outp/OverrideAndLimit  SystemSampleTime=-1  VariantActivationTime=update diagram  Latency=0  AutoFrameSizeCalculation=off
      link override Signal_Limit/_maxval: Value=KOUTP_HWVer3_cnt_maxval
      link override Signal_Limit/_minval: Value=KOUTP_HWVer3_cnt_minval
      link override Signal_Override/_ovrdflg: Value=KOUTP_HWVer3_cnt_ovrdflg
      link override Signal_Override/_ovrdval: Value=KOUTP_HWVer3_cnt_ovrdval
  VSYS_Major1_cnt_Inproc : FVT_lib/outp/OverrideAndLimit  SystemSampleTime=-1  VariantActivationTime=update diagram  Latency=0  AutoFrameSizeCalculation=off
      link override Signal_Limit/_maxval: Value=KOUTP_Major1_cnt_maxval
      link override Signal_Limit/_minval: Value=KOUTP_Major1_cnt_minval
      link override Signal_Override/_ovrdflg: Value=KOUTP_Major1_cnt_ovrdflg
      link override Signal_Override/_ovrdval: Value=KOUTP_Major1_cnt_ovrdval
  VSYS_Major2_cnt_Inproc : FVT_lib/outp/OverrideAndLimit  SystemSampleTime=-1  VariantActivationTime=update diagram  Latency=0  AutoFrameSizeCalculation=off
      link override Signal_Limit/_maxval: Value=KOUTP_Major2_cnt_maxval
      link override Signal_Limit/_minval: Value=KOUTP_Major2_cnt_minval
      link override Signal_Override/_ovrdflg: Value=KOUTP_Major2_cnt_ovrdflg
      link override Signal_Override/_ovrdval: Value=KOUTP_Major2_cnt_ovrdval
  VSYS_Minor1_cnt_Inproc : FVT_lib/outp/OverrideAndLimit  SystemSampleTime=-1  VariantActivationTime=update diagram  Latency=0  AutoFrameSizeCalculation=off
      link override Signal_Limit/_maxval: Value=KOUTP_Minor1_cnt_maxval
      link override Signal_Limit/_minval: Value=KOUTP_Minor1_cnt_minval
      link override Signal_Override/_ovrdflg: Value=KOUTP_Minor1_cnt_ovrdflg
      link override Signal_Override/_ovrdval: Value=KOUTP_Minor1_cnt_ovrdval
  VSYS_Minor2_cnt_Inproc : FVT_lib/outp/OverrideAndLimit  SystemSampleTime=-1  VariantActivationTime=update diagram  Latency=0  AutoFrameSizeCalculation=off
      link override Signal_Limit/_maxval: Value=KOUTP_Minor2_cnt_maxval
      link override Signal_Limit/_minval: Value=KOUTP_Minor2_cnt_minval
      link override Signal_Override/_ovrdflg: Value=KOUTP_Minor2_cnt_ovrdflg
      link override Signal_Override/_ovrdval: Value=KOUTP_Minor2_cnt_ovrdval
  VSYS_ModelYear_cnt_Inproc : FVT_lib/outp/OverrideAndLimit  SystemSampleTime=-1  VariantActivationTime=update diagram  Latency=0  AutoFrameSizeCalculation=off
      link override Signal_Limit/_maxval: Value=KOUTP_ModelYear_cnt_maxval
      link override Signal_Limit/_minval: Value=KOUTP_ModelYear_cnt_minval
      link override Signal_Override/_ovrdflg: Value=KOUTP_ModelYear_cnt_ovrdflg
      link override Signal_Override/_ovrdval: Value=KOUTP_ModelYear_cnt_ovrdval
  VSYS_NvWriteReqRisingEdge_flg_Inproc : FVT_lib/outp/OverrideAndLimit  SystemSampleTime=-1  VariantActivationTime=update diagram  Latency=0  AutoFrameSizeCalculation=off
      link override Signal_Limit/_maxval: Value=KOUTP_NvWriteReqRisingEdge_flg_maxval
      link override Signal_Limit/_minval: Value=KOUTP_NvWriteReqRisingEdge_flg_minval
      link override Signal_Override/_ovrdflg: Value=KOUTP_NvWriteReqRisingEdge_flg_ovrdflg
      link override Signal_Override/_ovrdval: Value=KOUTP_NvWriteReqRisingEdge_flg_ovrdval
  VSYS_Patch1_cnt_Inproc : FVT_lib/outp/OverrideAndLimit  SystemSampleTime=-1  VariantActivationTime=update diagram  Latency=0  AutoFrameSizeCalculation=off
      link override Signal_Limit/_maxval: Value=KOUTP_Patch1_cnt_maxval
      link override Signal_Limit/_minval: Value=KOUTP_Patch1_cnt_minval
      link override Signal_Override/_ovrdflg: Value=KOUTP_Patch1_cnt_ovrdflg
      link override Signal_Override/_ovrdval: Value=KOUTP_Patch1_cnt_ovrdval
  VSYS_Patch2_cnt_Inproc : FVT_lib/outp/OverrideAndLimit  SystemSampleTime=-1  VariantActivationTime=update diagram  Latency=0  AutoFrameSizeCalculation=off
      link override Signal_Limit/_maxval: Value=KOUTP_Patch2_cnt_maxval
      link override Signal_Limit/_minval: Value=KOUTP_Patch2_cnt_minval
      link override Signal_Override/_ovrdflg: Value=KOUTP_Patch2_cnt_ovrdflg
      link override Signal_Override/_ovrdval: Value=KOUTP_Patch2_cnt_ovrdval
  VSYS_PmicBootPath_raw32_Inproc : FVT_lib/outp/OverrideAndLimit  SystemSampleTime=-1  VariantActivationTime=update diagram  Latency=0  AutoFrameSizeCalculation=off
      link override Signal_Limit/_maxval: Value=KOUTP_PmicBootPath_raw32_maxval
      link override Signal_Limit/_minval: Value=KOUTP_PmicBootPath_raw32_minval
      link override Signal_Override/_ovrdflg: Value=KOUTP_PmicBootPath_raw32_ovrdflg
      link override Signal_Override/_ovrdval: Value=KOUTP_PmicBootPath_raw32_ovrdval
  VSYS_PmicBootReason_enum_Inproc : FVT_lib/outp/OverrideAndLimit  SystemSampleTime=-1  VariantActivationTime=update diagram  Latency=0  AutoFrameSizeCalculation=off
      link override Signal_Limit/_maxval: Value=KOUTP_PmicBootReason_enum_maxval
      link override Signal_Limit/_minval: Value=KOUTP_PmicBootReason_enum_minval
      link override Signal_Override/_ovrdflg: Value=KOUTP_PmicBootReason_enum_ovrdflg
      link override Signal_Override/_ovrdval: Value=KOUTP_PmicBootReason_enum_ovrdval
  VSYS_SHA1_cnt_Inproc : FVT_lib/outp/OverrideAndLimit  SystemSampleTime=-1  VariantActivationTime=update diagram  Latency=0  AutoFrameSizeCalculation=off
      link override Signal_Limit/_maxval: Value=KOUTP_SHA1_cnt_maxval
      link override Signal_Limit/_minval: Value=KOUTP_SHA1_cnt_minval
      link override Signal_Override/_ovrdflg: Value=KOUTP_SHA1_cnt_ovrdflg
      link override Signal_Override/_ovrdval: Value=KOUTP_SHA1_cnt_ovrdval
  VSYS_SHA2_cnt_Inproc : FVT_lib/outp/OverrideAndLimit  SystemSampleTime=-1  VariantActivationTime=update diagram  Latency=0  AutoFrameSizeCalculation=off
      link override Signal_Limit/_maxval: Value=KOUTP_SHA2_cnt_maxval
      link override Signal_Limit/_minval: Value=KOUTP_SHA2_cnt_minval
      link override Signal_Override/_ovrdflg: Value=KOUTP_SHA2_cnt_ovrdflg
      link override Signal_Override/_ovrdval: Value=KOUTP_SHA2_cnt_ovrdval
  VSYS_SHA3_cnt_Inproc : FVT_lib/outp/OverrideAndLimit  SystemSampleTime=-1  VariantActivationTime=update diagram  Latency=0  AutoFrameSizeCalculation=off
      link override Signal_Limit/_maxval: Value=KOUTP_SHA3_cnt_maxval
      link override Signal_Limit/_minval: Value=KOUTP_SHA3_cnt_minval
      link override Signal_Override/_ovrdflg: Value=KOUTP_SHA3_cnt_ovrdflg
      link override Signal_Override/_ovrdval: Value=KOUTP_SHA3_cnt_ovrdval
  VSYS_SHA4_cnt_Inproc : FVT_lib/outp/OverrideAndLimit  SystemSampleTime=-1  VariantActivationTime=update diagram  Latency=0  AutoFrameSizeCalculation=off
      link override Signal_Limit/_maxval: Value=KOUTP_SHA4_cnt_maxval
      link override Signal_Limit/_minval: Value=KOUTP_SHA4_cnt_minval
      link override Signal_Override/_ovrdflg: Value=KOUTP_SHA4_cnt_ovrdflg
      link override Signal_Override/_ovrdval: Value=KOUTP_SHA4_cnt_ovrdval
  VSYS_SHA5_cnt_Inproc : FVT_lib/outp/OverrideAndLimit  SystemSampleTime=-1  VariantActivationTime=update diagram  Latency=0  AutoFrameSizeCalculation=off
      link override Signal_Limit/_maxval: Value=KOUTP_SHA5_cnt_maxval
      link override Signal_Limit/_minval: Value=KOUTP_SHA5_cnt_minval
      link override Signal_Override/_ovrdflg: Value=KOUTP_SHA5_cnt_ovrdflg
      link override Signal_Override/_ovrdval: Value=KOUTP_SHA5_cnt_ovrdval
  VSYS_SHA6_cnt_Inproc : FVT_lib/outp/OverrideAndLimit  SystemSampleTime=-1  VariantActivationTime=update diagram  Latency=0  AutoFrameSizeCalculation=off
      link override Signal_Limit/_maxval: Value=KOUTP_SHA6_cnt_maxval
      link override Signal_Limit/_minval: Value=KOUTP_SHA6_cnt_minval
      link override Signal_Override/_ovrdflg: Value=KOUTP_SHA6_cnt_ovrdflg
      link override Signal_Override/_ovrdval: Value=KOUTP_SHA6_cnt_ovrdval
  VSYS_SHA7_cnt_Inproc : FVT_lib/outp/OverrideAndLimit  SystemSampleTime=-1  VariantActivationTime=update diagram  Latency=0  AutoFrameSizeCalculation=off
      link override Signal_Limit/_maxval: Value=KOUTP_SHA7_cnt_maxval
      link override Signal_Limit/_minval: Value=KOUTP_SHA7_cnt_minval
      link override Signal_Override/_ovrdflg: Value=KOUTP_SHA7_cnt_ovrdflg
      link override Signal_Override/_ovrdval: Value=KOUTP_SHA7_cnt_ovrdval
  VSYS_SHA8_cnt_Inproc : FVT_lib/outp/OverrideAndLimit  SystemSampleTime=-1  VariantActivationTime=update diagram  Latency=0  AutoFrameSizeCalculation=off
      link override Signal_Limit/_maxval: Value=KOUTP_SHA8_cnt_maxval
      link override Signal_Limit/_minval: Value=KOUTP_SHA8_cnt_minval
      link override Signal_Override/_ovrdflg: Value=KOUTP_SHA8_cnt_ovrdflg
      link override Signal_Override/_ovrdval: Value=KOUTP_SHA8_cnt_ovrdval
  VSYS_Var4_cnt_Inproc : FVT_lib/outp/OverrideAndLimit  SystemSampleTime=-1  VariantActivationTime=update diagram  Latency=0  AutoFrameSizeCalculation=off
      link override Signal_Limit/_maxval: Value=KOUTP_Var4_cnt_maxval
      link override Signal_Limit/_minval: Value=KOUTP_Var4_cnt_minval
      link override Signal_Override/_ovrdflg: Value=KOUTP_Var4_cnt_ovrdflg
      link override Signal_Override/_ovrdval: Value=KOUTP_Var4_cnt_ovrdval
  VSYS_Var5_cnt_Inproc : FVT_lib/outp/OverrideAndLimit  SystemSampleTime=-1  VariantActivationTime=update diagram  Latency=0  AutoFrameSizeCalculation=off
      link override Signal_Limit/_maxval: Value=KOUTP_Var5_cnt_maxval
      link override Signal_Limit/_minval: Value=KOUTP_Var5_cnt_minval
      link override Signal_Override/_ovrdflg: Value=KOUTP_Var5_cnt_ovrdflg
      link override Signal_Override/_ovrdval: Value=KOUTP_Var5_cnt_ovrdval
  VSYS_Variation_cnt_Inproc : FVT_lib/outp/OverrideAndLimit  SystemSampleTime=-1  VariantActivationTime=update diagram  Latency=0  AutoFrameSizeCalculation=off
      link override Signal_Limit/_maxval: Value=KOUTP_Variation_cnt_maxval
      link override Signal_Limit/_minval: Value=KOUTP_Variation_cnt_minval
      link override Signal_Override/_ovrdflg: Value=KOUTP_Variation_cnt_ovrdflg
      link override Signal_Override/_ovrdval: Value=KOUTP_Variation_cnt_ovrdval
  VSYS_WisrBootReason_raw32_Inproc : FVT_lib/outp/OverrideAndLimit  SystemSampleTime=-1  VariantActivationTime=update diagram  Latency=0  AutoFrameSizeCalculation=off
      link override Signal_Limit/_maxval: Value=KOUTP_WisrBootReason_raw32_maxval
      link override Signal_Limit/_minval: Value=KOUTP_WisrBootReason_raw32_minval
      link override Signal_Override/_ovrdflg: Value=KOUTP_WisrBootReason_raw32_ovrdflg
      link override Signal_Override/_ovrdval: Value=KOUTP_WisrBootReason_raw32_ovrdval
  VTHC_ACModeMem_enum_Inproc : FVT_lib/outp/OverrideAndLimit  SystemSampleTime=-1  VariantActivationTime=update diagram  Latency=0  AutoFrameSizeCalculation=off
      link override Signal_Limit/_maxval: Value=KOUTP_ACModeMem_enum_maxval
      link override Signal_Limit/_minval: Value=KOUTP_ACModeMem_enum_minval
      link override Signal_Override/_ovrdflg: Value=KOUTP_ACModeMem_enum_ovrdflg
      link override Signal_Override/_ovrdval: Value=KOUTP_ACModeMem_enum_ovrdval
  VTHC_ACModeSet123_enum_Inproc : FVT_lib/outp/OverrideAndLimit  SystemSampleTime=-1  VariantActivationTime=update diagram  Latency=0  AutoFrameSizeCalculation=off
      link override Signal_Limit/_maxval: Value=KOUTP_ACModeSet123_enum_maxval
      link override Signal_Limit/_minval: Value=KOUTP_ACModeSet123_enum_minval
      link override Signal_Override/_ovrdflg: Value=KOUTP_ACModeSet123_enum_ovrdflg
      link override Signal_Override/_ovrdval: Value=KOUTP_ACModeSet123_enum_ovrdval
  VTHC_ACModeSet457_enum_Inproc : FVT_lib/outp/OverrideAndLimit  SystemSampleTime=-1  VariantActivationTime=update diagram  Latency=0  AutoFrameSizeCalculation=off
      link override Signal_Limit/_maxval: Value=KOUTP_ACModeSet457_enum_maxval
      link override Signal_Limit/_minval: Value=KOUTP_ACModeSet457_enum_minval
      link override Signal_Override/_ovrdflg: Value=KOUTP_ACModeSet457_enum_ovrdflg
      link override Signal_Override/_ovrdval: Value=KOUTP_ACModeSet457_enum_ovrdval
  VTHC_ACSubMode_enum_Inproc : FVT_lib/outp/OverrideAndLimit  SystemSampleTime=-1  VariantActivationTime=update diagram  Latency=0  AutoFrameSizeCalculation=off
      link override Signal_Limit/_maxval: Value=KOUTP_ACSubMode_enum_maxval
      link override Signal_Limit/_minval: Value=KOUTP_ACSubMode_enum_minval
      link override Signal_Override/_ovrdflg: Value=KOUTP_ACSubMode_enum_ovrdflg
      link override Signal_Override/_ovrdval: Value=KOUTP_ACSubMode_enum_ovrdval
  VTHC_AirIntenZone1MSet1_enum_Inproc : FVT_lib/outp/OverrideAndLimit  SystemSampleTime=-1  VariantActivationTime=update diagram  Latency=0  AutoFrameSizeCalculation=off
      link override Signal_Limit/_maxval: Value=KOUTP_AirIntenZone1MSet1_enum_maxval
      link override Signal_Limit/_minval: Value=KOUTP_AirIntenZone1MSet1_enum_minval
      link override Signal_Override/_ovrdflg: Value=KOUTP_AirIntenZone1MSet1_enum_ovrdflg
      link override Signal_Override/_ovrdval: Value=KOUTP_AirIntenZone1MSet1_enum_ovrdval
  VTHC_AirIntenZone1MSet2_enum_Inproc : FVT_lib/outp/OverrideAndLimit  SystemSampleTime=-1  VariantActivationTime=update diagram  Latency=0  AutoFrameSizeCalculation=off
      link override Signal_Limit/_maxval: Value=KOUTP_AirIntenZone1MSet2_enum_maxval
      link override Signal_Limit/_minval: Value=KOUTP_AirIntenZone1MSet2_enum_minval
      link override Signal_Override/_ovrdflg: Value=KOUTP_AirIntenZone1MSet2_enum_ovrdflg
      link override Signal_Override/_ovrdval: Value=KOUTP_AirIntenZone1MSet2_enum_ovrdval
  VTHC_AirIntenZone1MSet3_enum_Inproc : FVT_lib/outp/OverrideAndLimit  SystemSampleTime=-1  VariantActivationTime=update diagram  Latency=0  AutoFrameSizeCalculation=off
      link override Signal_Limit/_maxval: Value=KOUTP_AirIntenZone1MSet3_enum_maxval
      link override Signal_Limit/_minval: Value=KOUTP_AirIntenZone1MSet3_enum_minval
      link override Signal_Override/_ovrdflg: Value=KOUTP_AirIntenZone1MSet3_enum_ovrdflg
      link override Signal_Override/_ovrdval: Value=KOUTP_AirIntenZone1MSet3_enum_ovrdval
  VTHC_AirIntenZone1MSet4_enum_Inproc : FVT_lib/outp/OverrideAndLimit  SystemSampleTime=-1  VariantActivationTime=update diagram  Latency=0  AutoFrameSizeCalculation=off
      link override Signal_Limit/_maxval: Value=KOUTP_AirIntenZone1MSet4_enum_maxval
      link override Signal_Limit/_minval: Value=KOUTP_AirIntenZone1MSet4_enum_minval
      link override Signal_Override/_ovrdflg: Value=KOUTP_AirIntenZone1MSet4_enum_ovrdflg
      link override Signal_Override/_ovrdval: Value=KOUTP_AirIntenZone1MSet4_enum_ovrdval
  VTHC_AirIntenZone1MSet5_enum_Inproc : FVT_lib/outp/OverrideAndLimit  SystemSampleTime=-1  VariantActivationTime=update diagram  Latency=0  AutoFrameSizeCalculation=off
      link override Signal_Limit/_maxval: Value=KOUTP_AirIntenZone1MSet5_enum_maxval
      link override Signal_Limit/_minval: Value=KOUTP_AirIntenZone1MSet5_enum_minval
      link override Signal_Override/_ovrdflg: Value=KOUTP_AirIntenZone1MSet5_enum_ovrdflg
      link override Signal_Override/_ovrdval: Value=KOUTP_AirIntenZone1MSet5_enum_ovrdval
  VTHC_AirIntenZone1MSet7_enum_Inproc : FVT_lib/outp/OverrideAndLimit  SystemSampleTime=-1  VariantActivationTime=update diagram  Latency=0  AutoFrameSizeCalculation=off
      link override Signal_Limit/_maxval: Value=KOUTP_AirIntenZone1MSet7_enum_maxval
      link override Signal_Limit/_minval: Value=KOUTP_AirIntenZone1MSet7_enum_minval
      link override Signal_Override/_ovrdflg: Value=KOUTP_AirIntenZone1MSet7_enum_ovrdflg
      link override Signal_Override/_ovrdval: Value=KOUTP_AirIntenZone1MSet7_enum_ovrdval
  VTHC_AirIntenZone1M_enum_Inproc : FVT_lib/outp/OverrideAndLimit  SystemSampleTime=-1  VariantActivationTime=update diagram  Latency=0  AutoFrameSizeCalculation=off
      link override Signal_Limit/_maxval: Value=KOUTP_AirIntenZone1M_enum_maxval
      link override Signal_Limit/_minval: Value=KOUTP_AirIntenZone1M_enum_minval
      link override Signal_Override/_ovrdflg: Value=KOUTP_AirIntenZone1M_enum_ovrdflg
      link override Signal_Override/_ovrdval: Value=KOUTP_AirIntenZone1M_enum_ovrdval
  VTHC_AirIntenZone3MSet1_enum_Inproc : FVT_lib/outp/OverrideAndLimit  SystemSampleTime=-1  VariantActivationTime=update diagram  Latency=0  AutoFrameSizeCalculation=off
      link override Signal_Limit/_maxval: Value=KOUTP_AirIntenZone3MSet1_enum_maxval
      link override Signal_Limit/_minval: Value=KOUTP_AirIntenZone3MSet1_enum_minval
      link override Signal_Override/_ovrdflg: Value=KOUTP_AirIntenZone3MSet1_enum_ovrdflg
      link override Signal_Override/_ovrdval: Value=KOUTP_AirIntenZone3MSet1_enum_ovrdval
  VTHC_AirIntenZone3MSet2_enum_Inproc : FVT_lib/outp/OverrideAndLimit  SystemSampleTime=-1  VariantActivationTime=update diagram  Latency=0  AutoFrameSizeCalculation=off
      link override Signal_Limit/_maxval: Value=KOUTP_AirIntenZone3MSet2_enum_maxval
      link override Signal_Limit/_minval: Value=KOUTP_AirIntenZone3MSet2_enum_minval
      link override Signal_Override/_ovrdflg: Value=KOUTP_AirIntenZone3MSet2_enum_ovrdflg
      link override Signal_Override/_ovrdval: Value=KOUTP_AirIntenZone3MSet2_enum_ovrdval
  VTHC_AirIntenZone3MSet3_enum_Inproc : FVT_lib/outp/OverrideAndLimit  SystemSampleTime=-1  VariantActivationTime=update diagram  Latency=0  AutoFrameSizeCalculation=off
      link override Signal_Limit/_maxval: Value=KOUTP_AirIntenZone3MSet3_enum_maxval
      link override Signal_Limit/_minval: Value=KOUTP_AirIntenZone3MSet3_enum_minval
      link override Signal_Override/_ovrdflg: Value=KOUTP_AirIntenZone3MSet3_enum_ovrdflg
      link override Signal_Override/_ovrdval: Value=KOUTP_AirIntenZone3MSet3_enum_ovrdval
  VTHC_AirIntenZone3MSet4_enum_Inproc : FVT_lib/outp/OverrideAndLimit  SystemSampleTime=-1  VariantActivationTime=update diagram  Latency=0  AutoFrameSizeCalculation=off
      link override Signal_Limit/_maxval: Value=KOUTP_AirIntenZone3MSet4_enum_maxval
      link override Signal_Limit/_minval: Value=KOUTP_AirIntenZone3MSet4_enum_minval
      link override Signal_Override/_ovrdflg: Value=KOUTP_AirIntenZone3MSet4_enum_ovrdflg
      link override Signal_Override/_ovrdval: Value=KOUTP_AirIntenZone3MSet4_enum_ovrdval
  VTHC_AirIntenZone3MSet5_enum_Inproc : FVT_lib/outp/OverrideAndLimit  SystemSampleTime=-1  VariantActivationTime=update diagram  Latency=0  AutoFrameSizeCalculation=off
      link override Signal_Limit/_maxval: Value=KOUTP_AirIntenZone3MSet5_enum_maxval
      link override Signal_Limit/_minval: Value=KOUTP_AirIntenZone3MSet5_enum_minval
      link override Signal_Override/_ovrdflg: Value=KOUTP_AirIntenZone3MSet5_enum_ovrdflg
      link override Signal_Override/_ovrdval: Value=KOUTP_AirIntenZone3MSet5_enum_ovrdval
  VTHC_AirIntenZone3MSet7_enum_Inproc : FVT_lib/outp/OverrideAndLimit  SystemSampleTime=-1  VariantActivationTime=update diagram  Latency=0  AutoFrameSizeCalculation=off
      link override Signal_Limit/_maxval: Value=KOUTP_AirIntenZone3MSet7_enum_maxval
      link override Signal_Limit/_minval: Value=KOUTP_AirIntenZone3MSet7_enum_minval
      link override Signal_Override/_ovrdflg: Value=KOUTP_AirIntenZone3MSet7_enum_ovrdflg
      link override Signal_Override/_ovrdval: Value=KOUTP_AirIntenZone3MSet7_enum_ovrdval
  VTHC_BatteryMode_enum_Inproc : FVT_lib/outp/OverrideAndLimit  SystemSampleTime=-1  VariantActivationTime=update diagram  Latency=0  AutoFrameSizeCalculation=off
      link override Signal_Limit/_maxval: Value=KOUTP_BatteryMode_enum_maxval
      link override Signal_Limit/_minval: Value=KOUTP_BatteryMode_enum_minval
      link override Signal_Override/_ovrdflg: Value=KOUTP_BatteryMode_enum_ovrdflg
      link override Signal_Override/_ovrdval: Value=KOUTP_BatteryMode_enum_ovrdval
  VTHC_CCUACLampSts_flg_Inproc : FVT_lib/outp/OverrideAndLimit  SystemSampleTime=-1  VariantActivationTime=update diagram  Latency=0  AutoFrameSizeCalculation=off
      link override Signal_Limit/_maxval: Value=KOUTP_CCUACLampSts_flg_maxval
      link override Signal_Limit/_minval: Value=KOUTP_CCUACLampSts_flg_minval
      link override Signal_Override/_ovrdflg: Value=KOUTP_CCUACLampSts_flg_ovrdflg
      link override Signal_Override/_ovrdval: Value=KOUTP_CCUACLampSts_flg_ovrdval
  VTHC_CCUACMaxLampSts_flg_Inproc : FVT_lib/outp/OverrideAndLimit  SystemSampleTime=-1  VariantActivationTime=update diagram  Latency=0  AutoFrameSizeCalculation=off
      link override Signal_Limit/_maxval: Value=KOUTP_CCUACMaxLampSts_flg_maxval
      link override Signal_Limit/_minval: Value=KOUTP_CCUACMaxLampSts_flg_minval
      link override Signal_Override/_ovrdflg: Value=KOUTP_CCUACMaxLampSts_flg_ovrdflg
      link override Signal_Override/_ovrdval: Value=KOUTP_CCUACMaxLampSts_flg_ovrdval
  VTHC_CCUAutoLampSts_flg_Inproc : FVT_lib/outp/OverrideAndLimit  SystemSampleTime=-1  VariantActivationTime=update diagram  Latency=0  AutoFrameSizeCalculation=off
      link override Signal_Limit/_maxval: Value=KOUTP_CCUAutoLampSts_flg_maxval
      link override Signal_Limit/_minval: Value=KOUTP_CCUAutoLampSts_flg_minval
      link override Signal_Override/_ovrdflg: Value=KOUTP_CCUAutoLampSts_flg_ovrdflg
      link override Signal_Override/_ovrdval: Value=KOUTP_CCUAutoLampSts_flg_ovrdval
  VTHC_CCUSyncLampSts_flg_Inproc : FVT_lib/outp/OverrideAndLimit  SystemSampleTime=-1  VariantActivationTime=update diagram  Latency=0  AutoFrameSizeCalculation=off
      link override Signal_Limit/_maxval: Value=KOUTP_CCUSyncLampSts_flg_maxval
      link override Signal_Limit/_minval: Value=KOUTP_CCUSyncLampSts_flg_minval
      link override Signal_Override/_ovrdflg: Value=KOUTP_CCUSyncLampSts_flg_ovrdflg
      link override Signal_Override/_ovrdval: Value=KOUTP_CCUSyncLampSts_flg_ovrdval
  VTHC_CCUSyncStsSet_enum_Inproc : FVT_lib/outp/OverrideAndLimit  SystemSampleTime=-1  VariantActivationTime=update diagram  Latency=0  AutoFrameSizeCalculation=off
      link override Signal_Limit/_maxval: Value=KOUTP_CCUSyncStsSet_enum_maxval
      link override Signal_Limit/_minval: Value=KOUTP_CCUSyncStsSet_enum_minval
      link override Signal_Override/_ovrdflg: Value=KOUTP_CCUSyncStsSet_enum_ovrdflg
      link override Signal_Override/_ovrdval: Value=KOUTP_CCUSyncStsSet_enum_ovrdval
  VTHC_CCUSyncSts_flg_Inproc : FVT_lib/outp/OverrideAndLimit  SystemSampleTime=-1  VariantActivationTime=update diagram  Latency=0  AutoFrameSizeCalculation=off
      link override Signal_Limit/_maxval: Value=KOUTP_CCUSyncSts_flg_maxval
      link override Signal_Limit/_minval: Value=KOUTP_CCUSyncSts_flg_minval
      link override Signal_Override/_ovrdflg: Value=KOUTP_CCUSyncSts_flg_ovrdflg
      link override Signal_Override/_ovrdval: Value=KOUTP_CCUSyncSts_flg_ovrdval
  VTHC_CLVentENSet_enum_Inproc : FVT_lib/outp/OverrideAndLimit  SystemSampleTime=-1  VariantActivationTime=update diagram  Latency=0  AutoFrameSizeCalculation=off
      link override Signal_Limit/_maxval: Value=KOUTP_CLVentENSet_enum_maxval
      link override Signal_Limit/_minval: Value=KOUTP_CLVentENSet_enum_minval
      link override Signal_Override/_ovrdflg: Value=KOUTP_CLVentENSet_enum_ovrdflg
      link override Signal_Override/_ovrdval: Value=KOUTP_CLVentENSet_enum_ovrdval
  VTHC_CLVentEN_flg_Inproc : FVT_lib/outp/OverrideAndLimit  SystemSampleTime=-1  VariantActivationTime=update diagram  Latency=0  AutoFrameSizeCalculation=off
      link override Signal_Limit/_maxval: Value=KOUTP_CLVentEN_flg_maxval
      link override Signal_Limit/_minval: Value=KOUTP_CLVentEN_flg_minval
      link override Signal_Override/_ovrdflg: Value=KOUTP_CLVentEN_flg_ovrdflg
      link override Signal_Override/_ovrdval: Value=KOUTP_CLVentEN_flg_ovrdval
  VTHC_CRVentENSet_enum_Inproc : FVT_lib/outp/OverrideAndLimit  SystemSampleTime=-1  VariantActivationTime=update diagram  Latency=0  AutoFrameSizeCalculation=off
      link override Signal_Limit/_maxval: Value=KOUTP_CRVentENSet_enum_maxval
      link override Signal_Limit/_minval: Value=KOUTP_CRVentENSet_enum_minval
      link override Signal_Override/_ovrdflg: Value=KOUTP_CRVentENSet_enum_ovrdflg
      link override Signal_Override/_ovrdval: Value=KOUTP_CRVentENSet_enum_ovrdval
  VTHC_CRVentEN_flg_Inproc : FVT_lib/outp/OverrideAndLimit  SystemSampleTime=-1  VariantActivationTime=update diagram  Latency=0  AutoFrameSizeCalculation=off
      link override Signal_Limit/_maxval: Value=KOUTP_CRVentEN_flg_maxval
      link override Signal_Limit/_minval: Value=KOUTP_CRVentEN_flg_minval
      link override Signal_Override/_ovrdflg: Value=KOUTP_CRVentEN_flg_ovrdflg
      link override Signal_Override/_ovrdval: Value=KOUTP_CRVentEN_flg_ovrdval
  VTHC_CabinMode_enum_Inproc : FVT_lib/outp/OverrideAndLimit  SystemSampleTime=-1  VariantActivationTime=update diagram  Latency=0  AutoFrameSizeCalculation=off
      link override Signal_Limit/_maxval: Value=KOUTP_CabinMode_enum_maxval
      link override Signal_Limit/_minval: Value=KOUTP_CabinMode_enum_minval
      link override Signal_Override/_ovrdflg: Value=KOUTP_CabinMode_enum_ovrdflg
      link override Signal_Override/_ovrdval: Value=KOUTP_CabinMode_enum_ovrdval
  VTHC_CoolgFanActDuty_pct_Inproc : FVT_lib/outp/OverrideAndLimit  SystemSampleTime=-1  VariantActivationTime=update diagram  Latency=0  AutoFrameSizeCalculation=off
      link override Signal_Limit/_maxval: Value=KOUTP_CoolgFanActDuty_pct_maxval
      link override Signal_Limit/_minval: Value=KOUTP_CoolgFanActDuty_pct_minval
      link override Signal_Override/_ovrdflg: Value=KOUTP_CoolgFanActDuty_pct_ovrdflg
      link override Signal_Override/_ovrdval: Value=KOUTP_CoolgFanActDuty_pct_ovrdval
  VTHC_EDriveMode_enum_Inproc : FVT_lib/outp/OverrideAndLimit  SystemSampleTime=-1  VariantActivationTime=update diagram  Latency=0  AutoFrameSizeCalculation=off
      link override Signal_Limit/_maxval: Value=KOUTP_EDriveMode_enum_maxval
      link override Signal_Limit/_minval: Value=KOUTP_EDriveMode_enum_minval
      link override Signal_Override/_ovrdflg: Value=KOUTP_EDriveMode_enum_ovrdflg
      link override Signal_Override/_ovrdval: Value=KOUTP_EDriveMode_enum_ovrdval
  VTHC_EWPBUflag1_flg_Inproc : FVT_lib/outp/OverrideAndLimit  SystemSampleTime=-1  VariantActivationTime=update diagram  Latency=0  AutoFrameSizeCalculation=off
      link override Signal_Limit/_maxval: Value=KOUTP_EWPBUflag1_flg_maxval
      link override Signal_Limit/_minval: Value=KOUTP_EWPBUflag1_flg_minval
      link override Signal_Override/_ovrdflg: Value=KOUTP_EWPBUflag1_flg_ovrdflg
      link override Signal_Override/_ovrdval: Value=KOUTP_EWPBUflag1_flg_ovrdval
  VTHC_EWPBUflag2_flg_Inproc : FVT_lib/outp/OverrideAndLimit  SystemSampleTime=-1  VariantActivationTime=update diagram  Latency=0  AutoFrameSizeCalculation=off
      link override Signal_Limit/_maxval: Value=KOUTP_EWPBUflag2_flg_maxval
      link override Signal_Limit/_minval: Value=KOUTP_EWPBUflag2_flg_minval
      link override Signal_Override/_ovrdflg: Value=KOUTP_EWPBUflag2_flg_ovrdflg
      link override Signal_Override/_ovrdval: Value=KOUTP_EWPBUflag2_flg_ovrdval
  VTHC_EWPBUflag3_flg_Inproc : FVT_lib/outp/OverrideAndLimit  SystemSampleTime=-1  VariantActivationTime=update diagram  Latency=0  AutoFrameSizeCalculation=off
      link override Signal_Limit/_maxval: Value=KOUTP_EWPBUflag3_flg_maxval
      link override Signal_Limit/_minval: Value=KOUTP_EWPBUflag3_flg_minval
      link override Signal_Override/_ovrdflg: Value=KOUTP_EWPBUflag3_flg_ovrdflg
      link override Signal_Override/_ovrdval: Value=KOUTP_EWPBUflag3_flg_ovrdval
  VTHC_FACESet_enum_Inproc : FVT_lib/outp/OverrideAndLimit  SystemSampleTime=-1  VariantActivationTime=update diagram  Latency=0  AutoFrameSizeCalculation=off
      link override Signal_Limit/_maxval: Value=KOUTP_FACESet_enum_maxval
      link override Signal_Limit/_minval: Value=KOUTP_FACESet_enum_minval
      link override Signal_Override/_ovrdflg: Value=KOUTP_FACESet_enum_ovrdflg
      link override Signal_Override/_ovrdval: Value=KOUTP_FACESet_enum_ovrdval
  VTHC_FDAGSCmd_enum_Inproc : FVT_lib/outp/OverrideAndLimit  SystemSampleTime=-1  VariantActivationTime=update diagram  Latency=0  AutoFrameSizeCalculation=off
      link override Signal_Limit/_maxval: Value=KOUTP_FDAGSCmd_enum_maxval
      link override Signal_Limit/_minval: Value=KOUTP_FDAGSCmd_enum_minval
      link override Signal_Override/_ovrdflg: Value=KOUTP_FDAGSCmd_enum_ovrdflg
      link override Signal_Override/_ovrdval: Value=KOUTP_FDAGSCmd_enum_ovrdval
  VTHC_FDBlowerCmd_pct_Inproc : FVT_lib/outp/OverrideAndLimit  SystemSampleTime=-1  VariantActivationTime=update diagram  Latency=0  AutoFrameSizeCalculation=off
      link override Signal_Limit/_maxval: Value=KOUTP_FDBlowerCmd_pct_maxval
      link override Signal_Limit/_minval: Value=KOUTP_FDBlowerCmd_pct_minval
      link override Signal_Override/_ovrdflg: Value=KOUTP_FDBlowerCmd_pct_ovrdflg
      link override Signal_Override/_ovrdval: Value=KOUTP_FDBlowerCmd_pct_ovrdval
  VTHC_FDCFGSAirIntCmd_enum_Inproc : FVT_lib/outp/OverrideAndLimit  SystemSampleTime=-1  VariantActivationTime=update diagram  Latency=0  AutoFrameSizeCalculation=off
      link override Signal_Limit/_maxval: Value=KOUTP_FDCFGSAirIntCmd_enum_maxval
      link override Signal_Limit/_minval: Value=KOUTP_FDCFGSAirIntCmd_enum_minval
      link override Signal_Override/_ovrdflg: Value=KOUTP_FDCFGSAirIntCmd_enum_ovrdflg
      link override Signal_Override/_ovrdval: Value=KOUTP_FDCFGSAirIntCmd_enum_ovrdval
  VTHC_FDCFGSAirIntStaSet123_enum_Inproc : FVT_lib/outp/OverrideAndLimit  SystemSampleTime=-1  VariantActivationTime=update diagram  Latency=0  AutoFrameSizeCalculation=off
      link override Signal_Limit/_maxval: Value=KOUTP_FDCFGSAirIntStaSet123_enum_maxval
      link override Signal_Limit/_minval: Value=KOUTP_FDCFGSAirIntStaSet123_enum_minval
      link override Signal_Override/_ovrdflg: Value=KOUTP_FDCFGSAirIntStaSet123_enum_ovrdflg
      link override Signal_Override/_ovrdval: Value=KOUTP_FDCFGSAirIntStaSet123_enum_ovrdval
  VTHC_FDCFGSAirIntStaSet457_enum_Inproc : FVT_lib/outp/OverrideAndLimit  SystemSampleTime=-1  VariantActivationTime=update diagram  Latency=0  AutoFrameSizeCalculation=off
      link override Signal_Limit/_maxval: Value=KOUTP_FDCFGSAirIntStaSet457_enum_maxval
      link override Signal_Limit/_minval: Value=KOUTP_FDCFGSAirIntStaSet457_enum_minval
      link override Signal_Override/_ovrdflg: Value=KOUTP_FDCFGSAirIntStaSet457_enum_ovrdflg
      link override Signal_Override/_ovrdval: Value=KOUTP_FDCFGSAirIntStaSet457_enum_ovrdval
  VTHC_FDCFGSAirIntSta_enum_Inproc : FVT_lib/outp/OverrideAndLimit  SystemSampleTime=-1  VariantActivationTime=update diagram  Latency=0  AutoFrameSizeCalculation=off
      link override Signal_Limit/_maxval: Value=KOUTP_FDCFGSAirIntSta_enum_maxval
      link override Signal_Limit/_minval: Value=KOUTP_FDCFGSAirIntSta_enum_minval
      link override Signal_Override/_ovrdflg: Value=KOUTP_FDCFGSAirIntSta_enum_ovrdflg
      link override Signal_Override/_ovrdval: Value=KOUTP_FDCFGSAirIntSta_enum_ovrdval
  VTHC_FDCFGSChCmd_enum_Inproc : FVT_lib/outp/OverrideAndLimit  SystemSampleTime=-1  VariantActivationTime=update diagram  Latency=0  AutoFrameSizeCalculation=off
      link override Signal_Limit/_maxval: Value=KOUTP_FDCFGSChCmd_enum_maxval
      link override Signal_Limit/_minval: Value=KOUTP_FDCFGSChCmd_enum_minval
      link override Signal_Override/_ovrdflg: Value=KOUTP_FDCFGSChCmd_enum_ovrdflg
      link override Signal_Override/_ovrdval: Value=KOUTP_FDCFGSChCmd_enum_ovrdval
  VTHC_FDCFGSChStaSet123_enum_Inproc : FVT_lib/outp/OverrideAndLimit  SystemSampleTime=-1  VariantActivationTime=update diagram  Latency=0  AutoFrameSizeCalculation=off
      link override Signal_Limit/_maxval: Value=KOUTP_FDCFGSChStaSet123_enum_maxval
      link override Signal_Limit/_minval: Value=KOUTP_FDCFGSChStaSet123_enum_minval
      link override Signal_Override/_ovrdflg: Value=KOUTP_FDCFGSChStaSet123_enum_ovrdflg
      link override Signal_Override/_ovrdval: Value=KOUTP_FDCFGSChStaSet123_enum_ovrdval
  VTHC_FDCFGSChStaSet457_enum_Inproc : FVT_lib/outp/OverrideAndLimit  SystemSampleTime=-1  VariantActivationTime=update diagram  Latency=0  AutoFrameSizeCalculation=off
      link override Signal_Limit/_maxval: Value=KOUTP_FDCFGSChStaSet457_enum_maxval
      link override Signal_Limit/_minval: Value=KOUTP_FDCFGSChStaSet457_enum_minval
      link override Signal_Override/_ovrdflg: Value=KOUTP_FDCFGSChStaSet457_enum_ovrdflg
      link override Signal_Override/_ovrdval: Value=KOUTP_FDCFGSChStaSet457_enum_ovrdval
  VTHC_FDCFGSChSta_enum_Inproc : FVT_lib/outp/OverrideAndLimit  SystemSampleTime=-1  VariantActivationTime=update diagram  Latency=0  AutoFrameSizeCalculation=off
      link override Signal_Limit/_maxval: Value=KOUTP_FDCFGSChSta_enum_maxval
      link override Signal_Limit/_minval: Value=KOUTP_FDCFGSChSta_enum_minval
      link override Signal_Override/_ovrdflg: Value=KOUTP_FDCFGSChSta_enum_ovrdflg
      link override Signal_Override/_ovrdval: Value=KOUTP_FDCFGSChSta_enum_ovrdval
  VTHC_FDCFGSFuncSta_enum_Inproc : FVT_lib/outp/OverrideAndLimit  SystemSampleTime=-1  VariantActivationTime=update diagram  Latency=0  AutoFrameSizeCalculation=off
      link override Signal_Limit/_maxval: Value=KOUTP_FDCFGSFuncSta_enum_maxval
      link override Signal_Limit/_minval: Value=KOUTP_FDCFGSFuncSta_enum_minval
      link override Signal_Override/_ovrdflg: Value=KOUTP_FDCFGSFuncSta_enum_ovrdflg
      link override Signal_Override/_ovrdval: Value=KOUTP_FDCFGSFuncSta_enum_ovrdval
  VTHC_FDCFGSFuncSta_flg_Inproc : FVT_lib/outp/OverrideAndLimit  SystemSampleTime=-1  VariantActivationTime=update diagram  Latency=0  AutoFrameSizeCalculation=off
      link override Signal_Limit/_maxval: Value=KOUTP_FDCFGSFuncSta_flg_maxval
      link override Signal_Limit/_minval: Value=KOUTP_FDCFGSFuncSta_flg_minval
      link override Signal_Override/_ovrdflg: Value=KOUTP_FDCFGSFuncSta_flg_ovrdflg
      link override Signal_Override/_ovrdval: Value=KOUTP_FDCFGSFuncSta_flg_ovrdval
  VTHC_FDCFGSIONCmd_flg_Inproc : FVT_lib/outp/OverrideAndLimit  SystemSampleTime=-1  VariantActivationTime=update diagram  Latency=0  AutoFrameSizeCalculation=off
      link override Signal_Limit/_maxval: Value=KOUTP_FDCFGSIONCmd_flg_maxval
      link override Signal_Limit/_minval: Value=KOUTP_FDCFGSIONCmd_flg_minval
      link override Signal_Override/_ovrdflg: Value=KOUTP_FDCFGSIONCmd_flg_ovrdflg
      link override Signal_Override/_ovrdval: Value=KOUTP_FDCFGSIONCmd_flg_ovrdval
  VTHC_FDCFGSIONSWSta_flg_Inproc : FVT_lib/outp/OverrideAndLimit  SystemSampleTime=-1  VariantActivationTime=update diagram  Latency=0  AutoFrameSizeCalculation=off
      link override Signal_Limit/_maxval: Value=KOUTP_FDCFGSIONSWSta_flg_maxval
      link override Signal_Limit/_minval: Value=KOUTP_FDCFGSIONSWSta_flg_minval
      link override Signal_Override/_ovrdflg: Value=KOUTP_FDCFGSIONSWSta_flg_ovrdflg
      link override Signal_Override/_ovrdval: Value=KOUTP_FDCFGSIONSWSta_flg_ovrdval
  VTHC_FDCFGSLearnCmd_enum_Inproc : FVT_lib/outp/OverrideAndLimit  SystemSampleTime=-1  VariantActivationTime=update diagram  Latency=0  AutoFrameSizeCalculation=off
      link override Signal_Limit/_maxval: Value=KOUTP_FDCFGSLearnCmd_enum_maxval
      link override Signal_Limit/_minval: Value=KOUTP_FDCFGSLearnCmd_enum_minval
      link override Signal_Override/_ovrdflg: Value=KOUTP_FDCFGSLearnCmd_enum_ovrdflg
      link override Signal_Override/_ovrdval: Value=KOUTP_FDCFGSLearnCmd_enum_ovrdval
  VTHC_FDCTHCAirIntZ3Sta_enum_Inproc : FVT_lib/outp/OverrideAndLimit  SystemSampleTime=-1  VariantActivationTime=update diagram  Latency=0  AutoFrameSizeCalculation=off
      link override Signal_Limit/_maxval: Value=KOUTP_FDCTHCAirIntZ3Sta_enum_maxval
      link override Signal_Limit/_minval: Value=KOUTP_FDCTHCAirIntZ3Sta_enum_minval
      link override Signal_Override/_ovrdflg: Value=KOUTP_FDCTHCAirIntZ3Sta_enum_ovrdflg
      link override Signal_Override/_ovrdval: Value=KOUTP_FDCTHCAirIntZ3Sta_enum_ovrdval
  VTHC_FDCTHCCLEVentYStaSet1_enum_Inproc : FVT_lib/outp/OverrideAndLimit  SystemSampleTime=-1  VariantActivationTime=update diagram  Latency=0  AutoFrameSizeCalculation=off
      link override Signal_Limit/_maxval: Value=KOUTP_FDCTHCCLEVentYStaSet1_enum_maxval
      link override Signal_Limit/_minval: Value=KOUTP_FDCTHCCLEVentYStaSet1_enum_minval
      link override Signal_Override/_ovrdflg: Value=KOUTP_FDCTHCCLEVentYStaSet1_enum_ovrdflg
      link override Signal_Override/_ovrdval: Value=KOUTP_FDCTHCCLEVentYStaSet1_enum_ovrdval
  VTHC_FDCTHCCLEVentYStaSet2_enum_Inproc : FVT_lib/outp/OverrideAndLimit  SystemSampleTime=-1  VariantActivationTime=update diagram  Latency=0  AutoFrameSizeCalculation=off
      link override Signal_Limit/_maxval: Value=KOUTP_FDCTHCCLEVentYStaSet2_enum_maxval
      link override Signal_Limit/_minval: Value=KOUTP_FDCTHCCLEVentYStaSet2_enum_minval
      link override Signal_Override/_ovrdflg: Value=KOUTP_FDCTHCCLEVentYStaSet2_enum_ovrdflg
      link override Signal_Override/_ovrdval: Value=KOUTP_FDCTHCCLEVentYStaSet2_enum_ovrdval
  VTHC_FDCTHCCLEVentYStaSet3_enum_Inproc : FVT_lib/outp/OverrideAndLimit  SystemSampleTime=-1  VariantActivationTime=update diagram  Latency=0  AutoFrameSizeCalculation=off
      link override Signal_Limit/_maxval: Value=KOUTP_FDCTHCCLEVentYStaSet3_enum_maxval
      link override Signal_Limit/_minval: Value=KOUTP_FDCTHCCLEVentYStaSet3_enum_minval
      link override Signal_Override/_ovrdflg: Value=KOUTP_FDCTHCCLEVentYStaSet3_enum_ovrdflg
      link override Signal_Override/_ovrdval: Value=KOUTP_FDCTHCCLEVentYStaSet3_enum_ovrdval
  VTHC_FDCTHCCLEVentYStaSet4_enum_Inproc : FVT_lib/outp/OverrideAndLimit  SystemSampleTime=-1  VariantActivationTime=update diagram  Latency=0  AutoFrameSizeCalculation=off
      link override Signal_Limit/_maxval: Value=KOUTP_FDCTHCCLEVentYStaSet4_enum_maxval
      link override Signal_Limit/_minval: Value=KOUTP_FDCTHCCLEVentYStaSet4_enum_minval
      link override Signal_Override/_ovrdflg: Value=KOUTP_FDCTHCCLEVentYStaSet4_enum_ovrdflg
      link override Signal_Override/_ovrdval: Value=KOUTP_FDCTHCCLEVentYStaSet4_enum_ovrdval
  VTHC_FDCTHCCLEVentYStaSet5_enum_Inproc : FVT_lib/outp/OverrideAndLimit  SystemSampleTime=-1  VariantActivationTime=update diagram  Latency=0  AutoFrameSizeCalculation=off
      link override Signal_Limit/_maxval: Value=KOUTP_FDCTHCCLEVentYStaSet5_enum_maxval
      link override Signal_Limit/_minval: Value=KOUTP_FDCTHCCLEVentYStaSet5_enum_minval
      link override Signal_Override/_ovrdflg: Value=KOUTP_FDCTHCCLEVentYStaSet5_enum_ovrdflg
      link override Signal_Override/_ovrdval: Value=KOUTP_FDCTHCCLEVentYStaSet5_enum_ovrdval
  VTHC_FDCTHCCLEVentYStaSet7_enum_Inproc : FVT_lib/outp/OverrideAndLimit  SystemSampleTime=-1  VariantActivationTime=update diagram  Latency=0  AutoFrameSizeCalculation=off
      link override Signal_Limit/_maxval: Value=KOUTP_FDCTHCCLEVentYStaSet7_enum_maxval
      link override Signal_Limit/_minval: Value=KOUTP_FDCTHCCLEVentYStaSet7_enum_minval
      link override Signal_Override/_ovrdflg: Value=KOUTP_FDCTHCCLEVentYStaSet7_enum_ovrdflg
      link override Signal_Override/_ovrdval: Value=KOUTP_FDCTHCCLEVentYStaSet7_enum_ovrdval
  VTHC_FDCTHCCLEVentYSta_enum_Inproc : FVT_lib/outp/OverrideAndLimit  SystemSampleTime=-1  VariantActivationTime=update diagram  Latency=0  AutoFrameSizeCalculation=off
      link override Signal_Limit/_maxval: Value=KOUTP_FDCTHCCLEVentYSta_enum_maxval
      link override Signal_Limit/_minval: Value=KOUTP_FDCTHCCLEVentYSta_enum_minval
      link override Signal_Override/_ovrdflg: Value=KOUTP_FDCTHCCLEVentYSta_enum_ovrdflg
      link override Signal_Override/_ovrdval: Value=KOUTP_FDCTHCCLEVentYSta_enum_ovrdval
  VTHC_FDCTHCCLEVentZStaSet1_enum_Inproc : FVT_lib/outp/OverrideAndLimit  SystemSampleTime=-1  VariantActivationTime=update diagram  Latency=0  AutoFrameSizeCalculation=off
      link override Signal_Limit/_maxval: Value=KOUTP_FDCTHCCLEVentZStaSet1_enum_maxval
      link override Signal_Limit/_minval: Value=KOUTP_FDCTHCCLEVentZStaSet1_enum_minval
      link override Signal_Override/_ovrdflg: Value=KOUTP_FDCTHCCLEVentZStaSet1_enum_ovrdflg
      link override Signal_Override/_ovrdval: Value=KOUTP_FDCTHCCLEVentZStaSet1_enum_ovrdval
  VTHC_FDCTHCCLEVentZStaSet2_enum_Inproc : FVT_lib/outp/OverrideAndLimit  SystemSampleTime=-1  VariantActivationTime=update diagram  Latency=0  AutoFrameSizeCalculation=off
      link override Signal_Limit/_maxval: Value=KOUTP_FDCTHCCLEVentZStaSet2_enum_maxval
      link override Signal_Limit/_minval: Value=KOUTP_FDCTHCCLEVentZStaSet2_enum_minval
      link override Signal_Override/_ovrdflg: Value=KOUTP_FDCTHCCLEVentZStaSet2_enum_ovrdflg
      link override Signal_Override/_ovrdval: Value=KOUTP_FDCTHCCLEVentZStaSet2_enum_ovrdval
  VTHC_FDCTHCCLEVentZStaSet3_enum_Inproc : FVT_lib/outp/OverrideAndLimit  SystemSampleTime=-1  VariantActivationTime=update diagram  Latency=0  AutoFrameSizeCalculation=off
      link override Signal_Limit/_maxval: Value=KOUTP_FDCTHCCLEVentZStaSet3_enum_maxval
      link override Signal_Limit/_minval: Value=KOUTP_FDCTHCCLEVentZStaSet3_enum_minval
      link override Signal_Override/_ovrdflg: Value=KOUTP_FDCTHCCLEVentZStaSet3_enum_ovrdflg
      link override Signal_Override/_ovrdval: Value=KOUTP_FDCTHCCLEVentZStaSet3_enum_ovrdval
  VTHC_FDCTHCCLEVentZStaSet4_enum_Inproc : FVT_lib/outp/OverrideAndLimit  SystemSampleTime=-1  VariantActivationTime=update diagram  Latency=0  AutoFrameSizeCalculation=off
      link override Signal_Limit/_maxval: Value=KOUTP_FDCTHCCLEVentZStaSet4_enum_maxval
      link override Signal_Limit/_minval: Value=KOUTP_FDCTHCCLEVentZStaSet4_enum_minval
      link override Signal_Override/_ovrdflg: Value=KOUTP_FDCTHCCLEVentZStaSet4_enum_ovrdflg
      link override Signal_Override/_ovrdval: Value=KOUTP_FDCTHCCLEVentZStaSet4_enum_ovrdval
  VTHC_FDCTHCCLEVentZStaSet5_enum_Inproc : FVT_lib/outp/OverrideAndLimit  SystemSampleTime=-1  VariantActivationTime=update diagram  Latency=0  AutoFrameSizeCalculation=off
      link override Signal_Limit/_maxval: Value=KOUTP_FDCTHCCLEVentZStaSet5_enum_maxval
      link override Signal_Limit/_minval: Value=KOUTP_FDCTHCCLEVentZStaSet5_enum_minval
      link override Signal_Override/_ovrdflg: Value=KOUTP_FDCTHCCLEVentZStaSet5_enum_ovrdflg
      link override Signal_Override/_ovrdval: Value=KOUTP_FDCTHCCLEVentZStaSet5_enum_ovrdval
  VTHC_FDCTHCCLEVentZStaSet7_enum_Inproc : FVT_lib/outp/OverrideAndLimit  SystemSampleTime=-1  VariantActivationTime=update diagram  Latency=0  AutoFrameSizeCalculation=off
      link override Signal_Limit/_maxval: Value=KOUTP_FDCTHCCLEVentZStaSet7_enum_maxval
      link override Signal_Limit/_minval: Value=KOUTP_FDCTHCCLEVentZStaSet7_enum_minval
      link override Signal_Override/_ovrdflg: Value=KOUTP_FDCTHCCLEVentZStaSet7_enum_ovrdflg
      link override Signal_Override/_ovrdval: Value=KOUTP_FDCTHCCLEVentZStaSet7_enum_ovrdval
  VTHC_FDCTHCCLEVentZSta_enum_Inproc : FVT_lib/outp/OverrideAndLimit  SystemSampleTime=-1  VariantActivationTime=update diagram  Latency=0  AutoFrameSizeCalculation=off
      link override Signal_Limit/_maxval: Value=KOUTP_FDCTHCCLEVentZSta_enum_maxval
      link override Signal_Limit/_minval: Value=KOUTP_FDCTHCCLEVentZSta_enum_minval
      link override Signal_Override/_ovrdflg: Value=KOUTP_FDCTHCCLEVentZSta_enum_ovrdflg
      link override Signal_Override/_ovrdval: Value=KOUTP_FDCTHCCLEVentZSta_enum_ovrdval
  VTHC_FDCTHCCLVentENSta_flg_Inproc : FVT_lib/outp/OverrideAndLimit  SystemSampleTime=-1  VariantActivationTime=update diagram  Latency=0  AutoFrameSizeCalculation=off
      link override Signal_Limit/_maxval: Value=KOUTP_FDCTHCCLVentENSta_flg_maxval
      link override Signal_Limit/_minval: Value=KOUTP_FDCTHCCLVentENSta_flg_minval
      link override Signal_Override/_ovrdflg: Value=KOUTP_FDCTHCCLVentENSta_flg_ovrdflg
      link override Signal_Override/_ovrdval: Value=KOUTP_FDCTHCCLVentENSta_flg_ovrdval
  VTHC_FDCTHCCREVentYStaSet1_enum_Inproc : FVT_lib/outp/OverrideAndLimit  SystemSampleTime=-1  VariantActivationTime=update diagram  Latency=0  AutoFrameSizeCalculation=off
      link override Signal_Limit/_maxval: Value=KOUTP_FDCTHCCREVentYStaSet1_enum_maxval
      link override Signal_Limit/_minval: Value=KOUTP_FDCTHCCREVentYStaSet1_enum_minval
      link override Signal_Override/_ovrdflg: Value=KOUTP_FDCTHCCREVentYStaSet1_enum_ovrdflg
      link override Signal_Override/_ovrdval: Value=KOUTP_FDCTHCCREVentYStaSet1_enum_ovrdval
  VTHC_FDCTHCCREVentYStaSet2_enum_Inproc : FVT_lib/outp/OverrideAndLimit  SystemSampleTime=-1  VariantActivationTime=update diagram  Latency=0  AutoFrameSizeCalculation=off
      link override Signal_Limit/_maxval: Value=KOUTP_FDCTHCCREVentYStaSet2_enum_maxval
      link override Signal_Limit/_minval: Value=KOUTP_FDCTHCCREVentYStaSet2_enum_minval
      link override Signal_Override/_ovrdflg: Value=KOUTP_FDCTHCCREVentYStaSet2_enum_ovrdflg
      link override Signal_Override/_ovrdval: Value=KOUTP_FDCTHCCREVentYStaSet2_enum_ovrdval
  VTHC_FDCTHCCREVentYStaSet3_enum_Inproc : FVT_lib/outp/OverrideAndLimit  SystemSampleTime=-1  VariantActivationTime=update diagram  Latency=0  AutoFrameSizeCalculation=off
      link override Signal_Limit/_maxval: Value=KOUTP_FDCTHCCREVentYStaSet3_enum_maxval
      link override Signal_Limit/_minval: Value=KOUTP_FDCTHCCREVentYStaSet3_enum_minval
      link override Signal_Override/_ovrdflg: Value=KOUTP_FDCTHCCREVentYStaSet3_enum_ovrdflg
      link override Signal_Override/_ovrdval: Value=KOUTP_FDCTHCCREVentYStaSet3_enum_ovrdval
  VTHC_FDCTHCCREVentYStaSet4_enum_Inproc : FVT_lib/outp/OverrideAndLimit  SystemSampleTime=-1  VariantActivationTime=update diagram  Latency=0  AutoFrameSizeCalculation=off
      link override Signal_Limit/_maxval: Value=KOUTP_FDCTHCCREVentYStaSet4_enum_maxval
      link override Signal_Limit/_minval: Value=KOUTP_FDCTHCCREVentYStaSet4_enum_minval
      link override Signal_Override/_ovrdflg: Value=KOUTP_FDCTHCCREVentYStaSet4_enum_ovrdflg
      link override Signal_Override/_ovrdval: Value=KOUTP_FDCTHCCREVentYStaSet4_enum_ovrdval
  VTHC_FDCTHCCREVentYStaSet5_enum_Inproc : FVT_lib/outp/OverrideAndLimit  SystemSampleTime=-1  VariantActivationTime=update diagram  Latency=0  AutoFrameSizeCalculation=off
      link override Signal_Limit/_maxval: Value=KOUTP_FDCTHCCREVentYStaSet5_enum_maxval
      link override Signal_Limit/_minval: Value=KOUTP_FDCTHCCREVentYStaSet5_enum_minval
      link override Signal_Override/_ovrdflg: Value=KOUTP_FDCTHCCREVentYStaSet5_enum_ovrdflg
      link override Signal_Override/_ovrdval: Value=KOUTP_FDCTHCCREVentYStaSet5_enum_ovrdval
  VTHC_FDCTHCCREVentYStaSet7_enum_Inproc : FVT_lib/outp/OverrideAndLimit  SystemSampleTime=-1  VariantActivationTime=update diagram  Latency=0  AutoFrameSizeCalculation=off
      link override Signal_Limit/_maxval: Value=KOUTP_FDCTHCCREVentYStaSet7_enum_maxval
      link override Signal_Limit/_minval: Value=KOUTP_FDCTHCCREVentYStaSet7_enum_minval
      link override Signal_Override/_ovrdflg: Value=KOUTP_FDCTHCCREVentYStaSet7_enum_ovrdflg
      link override Signal_Override/_ovrdval: Value=KOUTP_FDCTHCCREVentYStaSet7_enum_ovrdval
  VTHC_FDCTHCCREVentYSta_enum_Inproc : FVT_lib/outp/OverrideAndLimit  SystemSampleTime=-1  VariantActivationTime=update diagram  Latency=0  AutoFrameSizeCalculation=off
      link override Signal_Limit/_maxval: Value=KOUTP_FDCTHCCREVentYSta_enum_maxval
      link override Signal_Limit/_minval: Value=KOUTP_FDCTHCCREVentYSta_enum_minval
      link override Signal_Override/_ovrdflg: Value=KOUTP_FDCTHCCREVentYSta_enum_ovrdflg
      link override Signal_Override/_ovrdval: Value=KOUTP_FDCTHCCREVentYSta_enum_ovrdval
  VTHC_FDCTHCCREVentZStaSet1_enum_Inproc : FVT_lib/outp/OverrideAndLimit  SystemSampleTime=-1  VariantActivationTime=update diagram  Latency=0  AutoFrameSizeCalculation=off
      link override Signal_Limit/_maxval: Value=KOUTP_FDCTHCCREVentZStaSet1_enum_maxval
      link override Signal_Limit/_minval: Value=KOUTP_FDCTHCCREVentZStaSet1_enum_minval
      link override Signal_Override/_ovrdflg: Value=KOUTP_FDCTHCCREVentZStaSet1_enum_ovrdflg
      link override Signal_Override/_ovrdval: Value=KOUTP_FDCTHCCREVentZStaSet1_enum_ovrdval
  VTHC_FDCTHCCREVentZStaSet2_enum_Inproc : FVT_lib/outp/OverrideAndLimit  SystemSampleTime=-1  VariantActivationTime=update diagram  Latency=0  AutoFrameSizeCalculation=off
      link override Signal_Limit/_maxval: Value=KOUTP_FDCTHCCREVentZStaSet2_enum_maxval
      link override Signal_Limit/_minval: Value=KOUTP_FDCTHCCREVentZStaSet2_enum_minval
      link override Signal_Override/_ovrdflg: Value=KOUTP_FDCTHCCREVentZStaSet2_enum_ovrdflg
      link override Signal_Override/_ovrdval: Value=KOUTP_FDCTHCCREVentZStaSet2_enum_ovrdval
  VTHC_FDCTHCCREVentZStaSet3_enum_Inproc : FVT_lib/outp/OverrideAndLimit  SystemSampleTime=-1  VariantActivationTime=update diagram  Latency=0  AutoFrameSizeCalculation=off
      link override Signal_Limit/_maxval: Value=KOUTP_FDCTHCCREVentZStaSet3_enum_maxval
      link override Signal_Limit/_minval: Value=KOUTP_FDCTHCCREVentZStaSet3_enum_minval
      link override Signal_Override/_ovrdflg: Value=KOUTP_FDCTHCCREVentZStaSet3_enum_ovrdflg
      link override Signal_Override/_ovrdval: Value=KOUTP_FDCTHCCREVentZStaSet3_enum_ovrdval
  VTHC_FDCTHCCREVentZStaSet4_enum_Inproc : FVT_lib/outp/OverrideAndLimit  SystemSampleTime=-1  VariantActivationTime=update diagram  Latency=0  AutoFrameSizeCalculation=off
      link override Signal_Limit/_maxval: Value=KOUTP_FDCTHCCREVentZStaSet4_enum_maxval
      link override Signal_Limit/_minval: Value=KOUTP_FDCTHCCREVentZStaSet4_enum_minval
      link override Signal_Override/_ovrdflg: Value=KOUTP_FDCTHCCREVentZStaSet4_enum_ovrdflg
      link override Signal_Override/_ovrdval: Value=KOUTP_FDCTHCCREVentZStaSet4_enum_ovrdval
  VTHC_FDCTHCCREVentZStaSet5_enum_Inproc : FVT_lib/outp/OverrideAndLimit  SystemSampleTime=-1  VariantActivationTime=update diagram  Latency=0  AutoFrameSizeCalculation=off
      link override Signal_Limit/_maxval: Value=KOUTP_FDCTHCCREVentZStaSet5_enum_maxval
      link override Signal_Limit/_minval: Value=KOUTP_FDCTHCCREVentZStaSet5_enum_minval
      link override Signal_Override/_ovrdflg: Value=KOUTP_FDCTHCCREVentZStaSet5_enum_ovrdflg
      link override Signal_Override/_ovrdval: Value=KOUTP_FDCTHCCREVentZStaSet5_enum_ovrdval
  VTHC_FDCTHCCREVentZStaSet7_enum_Inproc : FVT_lib/outp/OverrideAndLimit  SystemSampleTime=-1  VariantActivationTime=update diagram  Latency=0  AutoFrameSizeCalculation=off
      link override Signal_Limit/_maxval: Value=KOUTP_FDCTHCCREVentZStaSet7_enum_maxval
      link override Signal_Limit/_minval: Value=KOUTP_FDCTHCCREVentZStaSet7_enum_minval
      link override Signal_Override/_ovrdflg: Value=KOUTP_FDCTHCCREVentZStaSet7_enum_ovrdflg
      link override Signal_Override/_ovrdval: Value=KOUTP_FDCTHCCREVentZStaSet7_enum_ovrdval
  VTHC_FDCTHCCREVentZSta_enum_Inproc : FVT_lib/outp/OverrideAndLimit  SystemSampleTime=-1  VariantActivationTime=update diagram  Latency=0  AutoFrameSizeCalculation=off
      link override Signal_Limit/_maxval: Value=KOUTP_FDCTHCCREVentZSta_enum_maxval
      link override Signal_Limit/_minval: Value=KOUTP_FDCTHCCREVentZSta_enum_minval
      link override Signal_Override/_ovrdflg: Value=KOUTP_FDCTHCCREVentZSta_enum_ovrdflg
      link override Signal_Override/_ovrdval: Value=KOUTP_FDCTHCCREVentZSta_enum_ovrdval
  VTHC_FDCTHCCRVentENSta_flg_Inproc : FVT_lib/outp/OverrideAndLimit  SystemSampleTime=-1  VariantActivationTime=update diagram  Latency=0  AutoFrameSizeCalculation=off
      link override Signal_Limit/_maxval: Value=KOUTP_FDCTHCCRVentENSta_flg_maxval
      link override Signal_Limit/_minval: Value=KOUTP_FDCTHCCRVentENSta_flg_minval
      link override Signal_Override/_ovrdflg: Value=KOUTP_FDCTHCCRVentENSta_flg_ovrdflg
      link override Signal_Override/_ovrdval: Value=KOUTP_FDCTHCCRVentENSta_flg_ovrdval
  VTHC_FDCTHCLEVentModeSta_enum_Inproc : FVT_lib/outp/OverrideAndLimit  SystemSampleTime=-1  VariantActivationTime=update diagram  Latency=0  AutoFrameSizeCalculation=off
      link override Signal_Limit/_maxval: Value=KOUTP_FDCTHCLEVentModeSta_enum_maxval
      link override Signal_Limit/_minval: Value=KOUTP_FDCTHCLEVentModeSta_enum_minval
      link override Signal_Override/_ovrdflg: Value=KOUTP_FDCTHCLEVentModeSta_enum_ovrdflg
      link override Signal_Override/_ovrdval: Value=KOUTP_FDCTHCLEVentModeSta_enum_ovrdval
  VTHC_FDCTHCLEVentYStaSet1_enum_Inproc : FVT_lib/outp/OverrideAndLimit  SystemSampleTime=-1  VariantActivationTime=update diagram  Latency=0  AutoFrameSizeCalculation=off
      link override Signal_Limit/_maxval: Value=KOUTP_FDCTHCLEVentYStaSet1_enum_maxval
      link override Signal_Limit/_minval: Value=KOUTP_FDCTHCLEVentYStaSet1_enum_minval
      link override Signal_Override/_ovrdflg: Value=KOUTP_FDCTHCLEVentYStaSet1_enum_ovrdflg
      link override Signal_Override/_ovrdval: Value=KOUTP_FDCTHCLEVentYStaSet1_enum_ovrdval
  VTHC_FDCTHCLEVentYStaSet2_enum_Inproc : FVT_lib/outp/OverrideAndLimit  SystemSampleTime=-1  VariantActivationTime=update diagram  Latency=0  AutoFrameSizeCalculation=off
      link override Signal_Limit/_maxval: Value=KOUTP_FDCTHCLEVentYStaSet2_enum_maxval
      link override Signal_Limit/_minval: Value=KOUTP_FDCTHCLEVentYStaSet2_enum_minval
      link override Signal_Override/_ovrdflg: Value=KOUTP_FDCTHCLEVentYStaSet2_enum_ovrdflg
      link override Signal_Override/_ovrdval: Value=KOUTP_FDCTHCLEVentYStaSet2_enum_ovrdval
  VTHC_FDCTHCLEVentYStaSet3_enum_Inproc : FVT_lib/outp/OverrideAndLimit  SystemSampleTime=-1  VariantActivationTime=update diagram  Latency=0  AutoFrameSizeCalculation=off
      link override Signal_Limit/_maxval: Value=KOUTP_FDCTHCLEVentYStaSet3_enum_maxval
      link override Signal_Limit/_minval: Value=KOUTP_FDCTHCLEVentYStaSet3_enum_minval
      link override Signal_Override/_ovrdflg: Value=KOUTP_FDCTHCLEVentYStaSet3_enum_ovrdflg
      link override Signal_Override/_ovrdval: Value=KOUTP_FDCTHCLEVentYStaSet3_enum_ovrdval
  VTHC_FDCTHCLEVentYStaSet4_enum_Inproc : FVT_lib/outp/OverrideAndLimit  SystemSampleTime=-1  VariantActivationTime=update diagram  Latency=0  AutoFrameSizeCalculation=off
      link override Signal_Limit/_maxval: Value=KOUTP_FDCTHCLEVentYStaSet4_enum_maxval
      link override Signal_Limit/_minval: Value=KOUTP_FDCTHCLEVentYStaSet4_enum_minval
      link override Signal_Override/_ovrdflg: Value=KOUTP_FDCTHCLEVentYStaSet4_enum_ovrdflg
      link override Signal_Override/_ovrdval: Value=KOUTP_FDCTHCLEVentYStaSet4_enum_ovrdval
  VTHC_FDCTHCLEVentYStaSet5_enum_Inproc : FVT_lib/outp/OverrideAndLimit  SystemSampleTime=-1  VariantActivationTime=update diagram  Latency=0  AutoFrameSizeCalculation=off
      link override Signal_Limit/_maxval: Value=KOUTP_FDCTHCLEVentYStaSet5_enum_maxval
      link override Signal_Limit/_minval: Value=KOUTP_FDCTHCLEVentYStaSet5_enum_minval
      link override Signal_Override/_ovrdflg: Value=KOUTP_FDCTHCLEVentYStaSet5_enum_ovrdflg
      link override Signal_Override/_ovrdval: Value=KOUTP_FDCTHCLEVentYStaSet5_enum_ovrdval
  VTHC_FDCTHCLEVentYStaSet7_enum_Inproc : FVT_lib/outp/OverrideAndLimit  SystemSampleTime=-1  VariantActivationTime=update diagram  Latency=0  AutoFrameSizeCalculation=off
      link override Signal_Limit/_maxval: Value=KOUTP_FDCTHCLEVentYStaSet7_enum_maxval
      link override Signal_Limit/_minval: Value=KOUTP_FDCTHCLEVentYStaSet7_enum_minval
      link override Signal_Override/_ovrdflg: Value=KOUTP_FDCTHCLEVentYStaSet7_enum_ovrdflg
      link override Signal_Override/_ovrdval: Value=KOUTP_FDCTHCLEVentYStaSet7_enum_ovrdval
  VTHC_FDCTHCLEVentYSta_enum_Inproc : FVT_lib/outp/OverrideAndLimit  SystemSampleTime=-1  VariantActivationTime=update diagram  Latency=0  AutoFrameSizeCalculation=off
      link override Signal_Limit/_maxval: Value=KOUTP_FDCTHCLEVentYSta_enum_maxval
      link override Signal_Limit/_minval: Value=KOUTP_FDCTHCLEVentYSta_enum_minval
      link override Signal_Override/_ovrdflg: Value=KOUTP_FDCTHCLEVentYSta_enum_ovrdflg
      link override Signal_Override/_ovrdval: Value=KOUTP_FDCTHCLEVentYSta_enum_ovrdval
  VTHC_FDCTHCLEVentZStaSet1_enum_Inproc : FVT_lib/outp/OverrideAndLimit  SystemSampleTime=-1  VariantActivationTime=update diagram  Latency=0  AutoFrameSizeCalculation=off
      link override Signal_Limit/_maxval: Value=KOUTP_FDCTHCLEVentZStaSet1_enum_maxval
      link override Signal_Limit/_minval: Value=KOUTP_FDCTHCLEVentZStaSet1_enum_minval
      link override Signal_Override/_ovrdflg: Value=KOUTP_FDCTHCLEVentZStaSet1_enum_ovrdflg
      link override Signal_Override/_ovrdval: Value=KOUTP_FDCTHCLEVentZStaSet1_enum_ovrdval
  VTHC_FDCTHCLEVentZStaSet2_enum_Inproc : FVT_lib/outp/OverrideAndLimit  SystemSampleTime=-1  VariantActivationTime=update diagram  Latency=0  AutoFrameSizeCalculation=off
      link override Signal_Limit/_maxval: Value=KOUTP_FDCTHCLEVentZStaSet2_enum_maxval
      link override Signal_Limit/_minval: Value=KOUTP_FDCTHCLEVentZStaSet2_enum_minval
      link override Signal_Override/_ovrdflg: Value=KOUTP_FDCTHCLEVentZStaSet2_enum_ovrdflg
      link override Signal_Override/_ovrdval: Value=KOUTP_FDCTHCLEVentZStaSet2_enum_ovrdval
  VTHC_FDCTHCLEVentZStaSet3_enum_Inproc : FVT_lib/outp/OverrideAndLimit  SystemSampleTime=-1  VariantActivationTime=update diagram  Latency=0  AutoFrameSizeCalculation=off
      link override Signal_Limit/_maxval: Value=KOUTP_FDCTHCLEVentZStaSet3_enum_maxval
      link override Signal_Limit/_minval: Value=KOUTP_FDCTHCLEVentZStaSet3_enum_minval
      link override Signal_Override/_ovrdflg: Value=KOUTP_FDCTHCLEVentZStaSet3_enum_ovrdflg
      link override Signal_Override/_ovrdval: Value=KOUTP_FDCTHCLEVentZStaSet3_enum_ovrdval
  VTHC_FDCTHCLEVentZStaSet4_enum_Inproc : FVT_lib/outp/OverrideAndLimit  SystemSampleTime=-1  VariantActivationTime=update diagram  Latency=0  AutoFrameSizeCalculation=off
      link override Signal_Limit/_maxval: Value=KOUTP_FDCTHCLEVentZStaSet4_enum_maxval
      link override Signal_Limit/_minval: Value=KOUTP_FDCTHCLEVentZStaSet4_enum_minval
      link override Signal_Override/_ovrdflg: Value=KOUTP_FDCTHCLEVentZStaSet4_enum_ovrdflg
      link override Signal_Override/_ovrdval: Value=KOUTP_FDCTHCLEVentZStaSet4_enum_ovrdval
  VTHC_FDCTHCLEVentZStaSet5_enum_Inproc : FVT_lib/outp/OverrideAndLimit  SystemSampleTime=-1  VariantActivationTime=update diagram  Latency=0  AutoFrameSizeCalculation=off
      link override Signal_Limit/_maxval: Value=KOUTP_FDCTHCLEVentZStaSet5_enum_maxval
      link override Signal_Limit/_minval: Value=KOUTP_FDCTHCLEVentZStaSet5_enum_minval
      link override Signal_Override/_ovrdflg: Value=KOUTP_FDCTHCLEVentZStaSet5_enum_ovrdflg
      link override Signal_Override/_ovrdval: Value=KOUTP_FDCTHCLEVentZStaSet5_enum_ovrdval
  VTHC_FDCTHCLEVentZStaSet7_enum_Inproc : FVT_lib/outp/OverrideAndLimit  SystemSampleTime=-1  VariantActivationTime=update diagram  Latency=0  AutoFrameSizeCalculation=off
      link override Signal_Limit/_maxval: Value=KOUTP_FDCTHCLEVentZStaSet7_enum_maxval
      link override Signal_Limit/_minval: Value=KOUTP_FDCTHCLEVentZStaSet7_enum_minval
      link override Signal_Override/_ovrdflg: Value=KOUTP_FDCTHCLEVentZStaSet7_enum_ovrdflg
      link override Signal_Override/_ovrdval: Value=KOUTP_FDCTHCLEVentZStaSet7_enum_ovrdval
  VTHC_FDCTHCLEVentZSta_enum_Inproc : FVT_lib/outp/OverrideAndLimit  SystemSampleTime=-1  VariantActivationTime=update diagram  Latency=0  AutoFrameSizeCalculation=off
      link override Signal_Limit/_maxval: Value=KOUTP_FDCTHCLEVentZSta_enum_maxval
      link override Signal_Limit/_minval: Value=KOUTP_FDCTHCLEVentZSta_enum_minval
      link override Signal_Override/_ovrdflg: Value=KOUTP_FDCTHCLEVentZSta_enum_ovrdflg
      link override Signal_Override/_ovrdval: Value=KOUTP_FDCTHCLEVentZSta_enum_ovrdval
  VTHC_FDCTHCLVentENSta_flg_Inproc : FVT_lib/outp/OverrideAndLimit  SystemSampleTime=-1  VariantActivationTime=update diagram  Latency=0  AutoFrameSizeCalculation=off
      link override Signal_Limit/_maxval: Value=KOUTP_FDCTHCLVentENSta_flg_maxval
      link override Signal_Limit/_minval: Value=KOUTP_FDCTHCLVentENSta_flg_minval
      link override Signal_Override/_ovrdflg: Value=KOUTP_FDCTHCLVentENSta_flg_ovrdflg
      link override Signal_Override/_ovrdval: Value=KOUTP_FDCTHCLVentENSta_flg_ovrdval
  VTHC_FDCTHCMAPTCForceOFFSta_flg_Inproc : FVT_lib/outp/OverrideAndLimit  SystemSampleTime=-1  VariantActivationTime=update diagram  Latency=0  AutoFrameSizeCalculation=off
      link override Signal_Limit/_maxval: Value=KOUTP_FDCTHCMAPTCForceOFFSta_flg_maxval
      link override Signal_Limit/_minval: Value=KOUTP_FDCTHCMAPTCForceOFFSta_flg_minval
      link override Signal_Override/_ovrdflg: Value=KOUTP_FDCTHCMAPTCForceOFFSta_flg_ovrdflg
      link override Signal_Override/_ovrdval: Value=KOUTP_FDCTHCMAPTCForceOFFSta_flg_ovrdval
  VTHC_FDCTHCMPreWPTCHeatSta_enum_Inproc : FVT_lib/outp/OverrideAndLimit  SystemSampleTime=-1  VariantActivationTime=update diagram  Latency=0  AutoFrameSizeCalculation=off
      link override Signal_Limit/_maxval: Value=KOUTP_FDCTHCMPreWPTCHeatSta_enum_maxval
      link override Signal_Limit/_minval: Value=KOUTP_FDCTHCMPreWPTCHeatSta_enum_minval
      link override Signal_Override/_ovrdflg: Value=KOUTP_FDCTHCMPreWPTCHeatSta_enum_ovrdflg
      link override Signal_Override/_ovrdval: Value=KOUTP_FDCTHCMPreWPTCHeatSta_enum_ovrdval
  VTHC_FDCTHCREVentModeSta_enum_Inproc : FVT_lib/outp/OverrideAndLimit  SystemSampleTime=-1  VariantActivationTime=update diagram  Latency=0  AutoFrameSizeCalculation=off
      link override Signal_Limit/_maxval: Value=KOUTP_FDCTHCREVentModeSta_enum_maxval
      link override Signal_Limit/_minval: Value=KOUTP_FDCTHCREVentModeSta_enum_minval
      link override Signal_Override/_ovrdflg: Value=KOUTP_FDCTHCREVentModeSta_enum_ovrdflg
